simulink model "Heart_3D"  (R2024b)
settings: configuration reference "MasterConfig" (kept outside this file)
model workspace (MAT data in the model file):
  C_1 = 1
  C_10 = 23
  C_11 = 23
  C_12 = 23
  C_13 = 23
  C_14 = 23
  C_15 = 23
  C_16 = 23
  C_17 = 23
  C_18 = 23
  C_19 = 23
  C_2 = 1
  C_20 = 23
  C_21 = 23
  C_22 = 23
  C_23 = 2
  C_24 = 2
  C_25 = 2
  C_26 = 23
  C_27 = 23
  C_28 = 23
  C_29 = 23
  C_3 = 1
  C_30 = 50
  C_31 = 23
  C_32 = 23
  C_33 = 50
  C_34 = 23
  C_35 = 50
  C_36 = 23
  C_37 = 50
  C_38 = 50
  C_39 = 50
  C_4 = 1
  C_40 = 50
  C_41 = 50
  C_42 = 50
  C_43 = 50
  C_44 = 50
  C_45 = 23
  C_46 = 23
  C_47 = 23
  C_48 = 50
  C_49 = 50
  C_5 = 23
  C_50 = 23
  C_51 = 23
  C_52 = 23
  C_53 = 50
  C_54 = 50
  C_6 = 23
  C_7 = 23
  C_8 = 23
  C_9 = 23
  l_1 = 4.01400326634
  l_10 = 14.0362958077
  l_11 = 18.1950322891
  l_12 = 33.9599764429
  l_13 = 10
  l_14 = 8.0399004969
  l_15 = 12.0066648158
  l_16 = 7.69415362467
  l_17 = 5.21536192416
  l_18 = 5.65685424949
  l_19 = 13.8852439662
  l_2 = 3.2
  l_20 = 47.0387074652
  l_21 = 27.273430294
  l_22 = 13.8621787609
  l_23 = 18.6761880479
  l_24 = 12.8249756335
  l_25 = 15.879546593
  l_26 = 28.9689488936
  l_27 = 29.8073816361
  l_28 = 34.0352758179
  l_29 = 7.37563556583
  l_3 = 3.50907395191
  l_30 = 3.68781778292
  l_31 = 46.1042297409
  l_32 = 30.615028989
  l_33 = 7.51531769122
  l_34 = 7.47261667691
  l_35 = 3.73630833845
  l_36 = 36.7151195014
  l_37 = 16.1058995402
  l_38 = 48.7360236376
  l_39 = 48.8364617883
  l_4 = 4.54875807227
  l_40 = 41.4154560521
  l_41 = 37.7878287283
  l_42 = 44.689148571
  l_43 = 22.9120055866
  l_44 = 23.4401365184
  l_45 = 42.4264068712
  l_46 = 5
  l_47 = 8
  l_48 = 31.4273766007
  l_49 = 41.5788407727
  l_5 = 1.6986923075
  l_50 = 31.5569326773
  l_51 = 3
  l_52 = 3
  l_53 = 51.8478543433
  l_54 = 31.5569326773
  l_6 = 44.1540359298
  l_7 = 2.68208873828
  l_8 = 12.8
  l_9 = 4.53184289225
  xi_1 = 54.2
  xi_10 = 56.6
  xi_11 = 52.36
  xi_12 = 45
  xi_13 = 66.2
  xi_14 = 66.2
  xi_15 = 60.2
  xi_16 = 60.6
  xi_17 = 67
  xi_18 = 67.4
  xi_19 = 70.2
  xi_2 = 54.2
  xi_20 = 79.4
  xi_21 = 98.2
  xi_22 = 125.4
  xi_23 = 68.2
  xi_24 = 81.8
  xi_25 = 94.6
  xi_26 = 105
  xi_27 = 105
  xi_28 = 121.8
  xi_29 = 153
  xi_3 = 54.2
  xi_30 = 157.8
  xi_31 = 157.8
  xi_32 = 127.8
  xi_33 = 127.8
  xi_34 = 157
  xi_35 = 164.2
  xi_36 = 164.2
  xi_37 = 160.2
  xi_38 = 160.2
  xi_39 = 160.2
  xi_4 = 54.2
  xi_40 = 167.8
  xi_41 = 167.8
  xi_42 = 114.6
  xi_43 = 114.6
  xi_44 = 83
  xi_45 = 112.2
  xi_46 = 112.2
  xi_47 = 75
  xi_48 = 101.8
  xi_49 = 131
  xi_5 = 57.8666666667
  xi_50 = 159.4
  xi_51 = 159.4
  xi_52 = 143.4
  xi_53 = 112.2
  xi_54 = 162.4
  xi_6 = 57.8666666667
  xi_7 = 57.4
  xi_8 = 57.4
  xi_9 = 56.6
  xj_1 = 57.8666666667
  xj_10 = 66.2
  xj_11 = 45
  xj_12 = 53.8
  xj_13 = 60.2
  xj_14 = 67
  xj_15 = 60.6
  xj_16 = 68.2
  xj_17 = 67.4
  xj_18 = 68.2
  xj_19 = 79.4
  xj_2 = 57.4
  xj_20 = 118.6
  xj_21 = 125.4
  xj_22 = 135.4
  xj_23 = 81.8
  xj_24 = 94.6
  xj_25 = 105
  xj_26 = 121.8
  xj_27 = 127.8
  xj_28 = 153
  xj_29 = 157.8
  xj_3 = 56.6
  xj_30 = 160.2
  xj_31 = 112.2
  xj_32 = 157
  xj_33 = 131
  xj_34 = 164.2
  xj_35 = 167.8
  xj_36 = 159.4
  xj_37 = 167.8
  xj_38 = 114.6
  xj_39 = 112.2
  xj_4 = 52.36
  xj_40 = 131
  xj_41 = 162.4
  xj_42 = 83
  xj_43 = 131
  xj_44 = 101.8
  xj_45 = 75
  xj_46 = 112.2
  xj_47 = 67
  xj_48 = 125
  xj_49 = 101.8
  xj_5 = 57.4
  xj_50 = 143.4
  xj_51 = 162.4
  xj_52 = 146.4
  xj_53 = 67
  xj_54 = 146.4
  xj_6 = 98.2
  xj_7 = 56.6
  xj_8 = 70.2
  xj_9 = 52.36
  yi_1 = 118.2
  yi_10 = 115.64
  yi_11 = 114.04
  yi_12 = 97.4
  yi_13 = 105.4
  yi_14 = 105.4
  yi_15 = 97.4
  yi_16 = 85.4
  yi_17 = 97.4
  yi_18 = 92.2
  yi_19 = 118.2
  yi_2 = 118.2
  yi_20 = 107.8
  yi_21 = 137.8
  yi_22 = 139.8
  yi_23 = 86.6
  yi_24 = 99.4
  yi_25 = 100.2
  yi_26 = 88.2
  yi_27 = 88.2
  yi_28 = 64.6
  yi_29 = 51
  yi_3 = 118.2
  yi_30 = 45.4
  yi_31 = 45.4
  yi_32 = 69
  yi_33 = 69
  yi_34 = 59.8
  yi_35 = 57.8
  yi_36 = 57.8
  yi_37 = 42.6
  yi_38 = 42.6
  yi_39 = 42.6
  yi_4 = 118.2
  yi_40 = 56.8
  yi_41 = 56.8
  yi_42 = 59.8
  yi_43 = 59.8
  yi_44 = 91.4
  yi_45 = 38.6
  yi_46 = 38.6
  yi_47 = 59
  yi_48 = 105.4
  yi_49 = 75.8
  yi_5 = 119.833333333
  yi_50 = 94.2
  yi_51 = 94.2
  yi_52 = 121.4
  yi_53 = 33.6
  yi_54 = 94.2
  yi_6 = 119.833333333
  yi_7 = 118.2
  yi_8 = 118.2
  yi_9 = 115.64
  yj_1 = 119.833333333
  yj_10 = 105.4
  yj_11 = 97.4
  yj_12 = 64.6
  yj_13 = 97.4
  yj_14 = 97.4
  yj_15 = 85.4
  yj_16 = 86.6
  yj_17 = 92.2
  yj_18 = 86.6
  yj_19 = 107.8
  yj_2 = 118.2
  yj_20 = 133.8
  yj_21 = 139.8
  yj_22 = 130.2
  yj_23 = 99.4
  yj_24 = 100.2
  yj_25 = 88.2
  yj_26 = 64.6
  yj_27 = 69
  yj_28 = 51
  yj_29 = 45.4
  yj_3 = 115.64
  yj_30 = 42.6
  yj_31 = 38.6
  yj_32 = 59.8
  yj_33 = 75.8
  yj_34 = 57.8
  yj_35 = 56.8
  yj_36 = 94.2
  ... (+132 more variables)
undefined symbols (not defined in the file or in its folder): HeartCfg, Leads
(part 2 of 2)

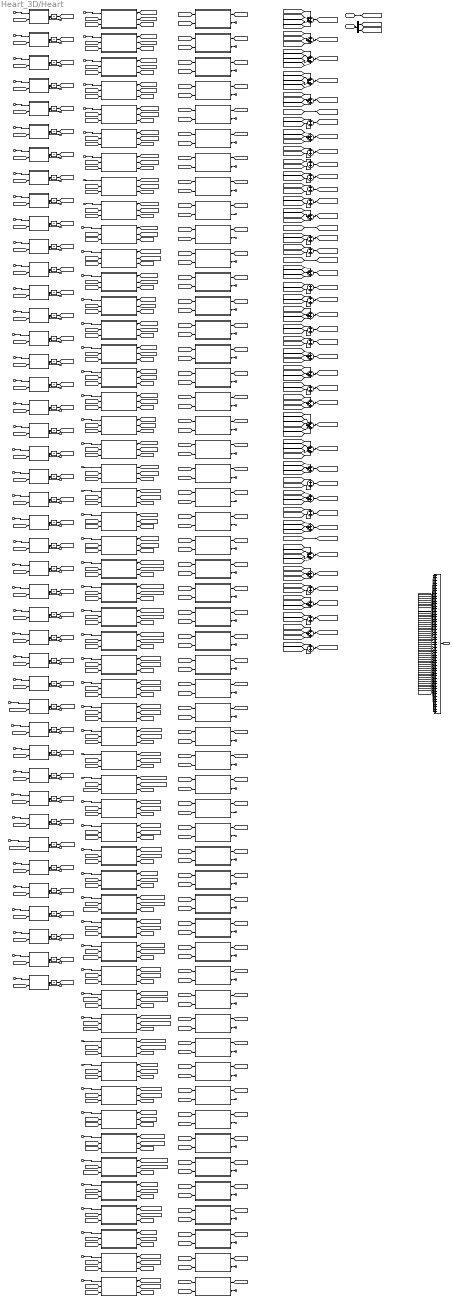
== system Heart_3D/Heart ==
  cfg_SA : Inport  PortName=cfg  Element=SA
  cfg_SA_a : Inport  PortName=cfg  Element=SA_a
  cfg_SA_b : Inport  PortName=cfg  Element=SA_b
  cfg_SA_c : Inport  PortName=cfg  Element=SA_c
  cfg_SA_d : Inport  PortName=cfg  Element=SA_d
  cfg_CT : Inport  PortName=cfg  Element=CT
  cfg_CT_a : Inport  PortName=cfg  Element=CT_a
  cfg_OS : Inport  PortName=cfg  Element=OS
  cfg_RE : Inport  PortName=cfg  Element=RE
  cfg_LNB : Inport  PortName=cfg  Element=LNB
  cfg_TC_f : Inport  PortName=cfg  Element=TC_f
  cfg_CN : Inport  PortName=cfg  Element=CN
  cfg_RA_a : Inport  PortName=cfg  Element=RA_a
  cfg_RA : Inport  PortName=cfg  Element=RA
  cfg_CS_LA : Inport  PortName=cfg  Element=CS_LA
  cfg_Bach : Inport  PortName=cfg  Element=Bach
  cfg_LA_a : Inport  PortName=cfg  Element=LA_a
  cfg_LA : Inport  PortName=cfg  Element=LA
  cfg_BH : Inport  PortName=cfg  Element=BH
  cfg_His_p : Inport  PortName=cfg  Element=His_p
  cfg_His_m : Inport  PortName=cfg  Element=His_m
  cfg_His_d : Inport  PortName=cfg  Element=His_d
  cfg_RBB_m : Inport  PortName=cfg  Element=RBB_m
  cfg_RBB : Inport  PortName=cfg  Element=RBB
  cfg_RBB_a : Inport  PortName=cfg  Element=RBB_a
  cfg_LBB_m : Inport  PortName=cfg  Element=LBB_m
  cfg_LBB : Inport  PortName=cfg  Element=LBB
  cfg_LBB_a : Inport  PortName=cfg  Element=LBB_a
  cfg_RVA : Inport  PortName=cfg  Element=RVA
  cfg_LVA : Inport  PortName=cfg  Element=LVA
  cfg_SEP_RV_m : Inport  PortName=cfg  Element=SEP_RV_m
  cfg_SEP_RV : Inport  PortName=cfg  Element=SEP_RV
  cfg_RV_m : Inport  PortName=cfg  Element=RV_m
  cfg_RV : Inport  PortName=cfg  Element=RV
  cfg_SEP_LV : Inport  PortName=cfg  Element=SEP_LV
  cfg_CS_LV : Inport  PortName=cfg  Element=CS_LV
  cfg_SEP_LV_m : Inport  PortName=cfg  Element=SEP_LV_m
  cfg_LV_m : Inport  PortName=cfg  Element=LV_m
  cfg_LV : Inport  PortName=cfg  Element=LV
  cfg_RV_mm : Inport  PortName=cfg  Element=RV_mm
  cfg_RVm : Inport  PortName=cfg  Element=RVm
  cfg_LV_mm : Inport  PortName=cfg  Element=LV_mm
  cfg_LVm : Inport  PortName=cfg  Element=LVm
  cfgPath_1_2 : Inport  PortName=cfg  Element=path_1
  cfgPath_1_3 : Inport  PortName=cfg  Element=path_2
  cfgPath_1_4 : Inport  PortName=cfg  Element=path_3
  cfgPath_1_5 : Inport  PortName=cfg  Element=path_4
  cfgPath_2_3 : Inport  PortName=cfg  Element=path_5
  cfgPath_2_16 : Inport  PortName=cfg  Element=path_6
  cfgPath_3_4 : Inport  PortName=cfg  Element=path_7
  cfgPath_3_13 : Inport  PortName=cfg  Element=path_8
  cfgPath_4_5 : Inport  PortName=cfg  Element=path_9
  cfgPath_4_8 : Inport  PortName=cfg  Element=path_10
  cfgPath_5_7 : Inport  PortName=cfg  Element=path_11
  cfgPath_6_7 : Inport  PortName=cfg  Element=path_12
  cfgPath_8_9 : Inport  PortName=cfg  Element=path_13
  cfgPath_8_11 : Inport  PortName=cfg  Element=path_14
  cfgPath_9_10 : Inport  PortName=cfg  Element=path_15
  cfgPath_10_19 : Inport  PortName=cfg  Element=path_16
  cfgPath_11_12 : Inport  PortName=cfg  Element=path_17
  cfgPath_12_19 : Inport  PortName=cfg  Element=path_18
  cfgPath_13_14 : Inport  PortName=cfg  Element=path_19
  cfgPath_14_15 : Inport  PortName=cfg  Element=path_20
  cfgPath_16_17 : Inport  PortName=cfg  Element=path_21
  cfgPath_17_18 : Inport  PortName=cfg  Element=path_22
  cfgPath_19_20 : Inport  PortName=cfg  Element=path_23
  cfgPath_20_21 : Inport  PortName=cfg  Element=path_24
  cfgPath_21_22 : Inport  PortName=cfg  Element=path_25
  cfgPath_22_23 : Inport  PortName=cfg  Element=path_26
  cfgPath_22_26 : Inport  PortName=cfg  Element=path_27
  cfgPath_23_24 : Inport  PortName=cfg  Element=path_28
  cfgPath_24_25 : Inport  PortName=cfg  Element=path_29
  cfgPath_25_29 : Inport  PortName=cfg  Element=path_30
  cfgPath_25_33 : Inport  PortName=cfg  Element=path_31
  cfgPath_26_27 : Inport  PortName=cfg  Element=path_32
  cfgPath_26_37 : Inport  PortName=cfg  Element=path_33
  cfgPath_27_28 : Inport  PortName=cfg  Element=path_34
  cfgPath_28_30 : Inport  PortName=cfg  Element=path_35
  cfgPath_28_38 : Inport  PortName=cfg  Element=path_36
  cfgPath_29_30 : Inport  PortName=cfg  Element=path_37
  cfgPath_29_31 : Inport  PortName=cfg  Element=path_38
  cfgPath_29_40 : Inport  PortName=cfg  Element=path_39
  cfgPath_30_37 : Inport  PortName=cfg  Element=path_40
  cfgPath_30_42 : Inport  PortName=cfg  Element=path_41
  cfgPath_31_32 : Inport  PortName=cfg  Element=path_42
  cfgPath_31_37 : Inport  PortName=cfg  Element=path_43
  cfgPath_32_35 : Inport  PortName=cfg  Element=path_44
  cfgPath_33_34 : Inport  PortName=cfg  Element=path_45
  cfgPath_33_40 : Inport  PortName=cfg  Element=path_46
  cfgPath_34_41 : Inport  PortName=cfg  Element=path_47
  cfgPath_35_36 : Inport  PortName=cfg  Element=path_48
  cfgPath_35_37 : Inport  PortName=cfg  Element=path_49
  cfgPath_38_39 : Inport  PortName=cfg  Element=path_50
  cfgPath_38_42 : Inport  PortName=cfg  Element=path_51
  cfgPath_39_43 : Inport  PortName=cfg  Element=path_52
  cfgPath_40_41 : Inport  PortName=cfg  Element=path_53
  cfgPath_42_43 : Inport  PortName=cfg  Element=path_54
  Leads : Inport  Port=2
  Pace : Inport  Port=3
  BH : ModelReference  ModelNameDialog=Node_NM  ModelReferenceVersion=1.97
  BH_His_p : ModelReference  ModelNameDialog=Path_model  ParameterArgumentNames=l  ParameterArgumentValues=l_23  UsingDefaultArgumentValue=0  ModelReferenceVersion=1.109
  BH_His_p_probe : ModelReference  ModelNameDialog=Electrode  UsingDefaultArgumentValue=0,0,0,0,0,0,0  ModelReferenceVersion=1.84
  Bach : ModelReference  ModelNameDialog=Node_M  ModelReferenceVersion=1.111
  Bach_LA_a : ModelReference  ModelNameDialog=Path_model  ParameterArgumentNames=l  ParameterArgumentValues=l_21  UsingDefaultArgumentValue=0  ModelReferenceVersion=1.109
  Bach_LA_a_probe : ModelReference  ModelNameDialog=Electrode  UsingDefaultArgumentValue=0,0,0,0,0,0,0  ModelReferenceVersion=1.84
  CN : ModelReference  ModelNameDialog=Node_N  ModelReferenceVersion=1.119
  CN_BH : ModelReference  ModelNameDialog=Path_model  ParameterArgumentNames=l  ParameterArgumentValues=l_18  UsingDefaultArgumentValue=0  ModelReferenceVersion=1.109
  CN_BH_probe : ModelReference  ModelNameDialog=Electrode  UsingDefaultArgumentValue=0,0,0,0,0,0,0  ModelReferenceVersion=1.84
  CS_LA : ModelReference  ModelNameDialog=Node_NM  ModelReferenceVersion=1.97
  CS_LV : ModelReference  ModelNameDialog=Node_M  ModelReferenceVersion=1.111
  CT : ModelReference  ModelNameDialog=Node_M  ModelReferenceVersion=1.111
  CT_CT_a : ModelReference  ModelNameDialog=Path_model  ParameterArgumentNames=l  ParameterArgumentValues=l_12  UsingDefaultArgumentValue=0  ModelReferenceVersion=1.109
  CT_CT_a_probe : ModelReference  ModelNameDialog=Electrode  UsingDefaultArgumentValue=0,0,0,0,0,0,0  ModelReferenceVersion=1.84
  CT_a : ModelReference  ModelNameDialog=Node_NM  ModelReferenceVersion=1.97
  CellDelay_BH : UnitDelay  SampleTime=-1  HasFrameUpgradeWarning=on
  CellDelay_Bach : UnitDelay  SampleTime=-1  HasFrameUpgradeWarning=on
  CellDelay_CN : UnitDelay  SampleTime=-1  HasFrameUpgradeWarning=on
  CellDelay_CS_LA : UnitDelay  SampleTime=-1  HasFrameUpgradeWarning=on
  CellDelay_CS_LV : UnitDelay  SampleTime=-1  HasFrameUpgradeWarning=on
  CellDelay_CT : UnitDelay  SampleTime=-1  HasFrameUpgradeWarning=on
  CellDelay_CT_a : UnitDelay  SampleTime=-1  HasFrameUpgradeWarning=on
  CellDelay_His_d : UnitDelay  SampleTime=-1  HasFrameUpgradeWarning=on
  CellDelay_His_m : UnitDelay  SampleTime=-1  HasFrameUpgradeWarning=on
  CellDelay_His_p : UnitDelay  SampleTime=-1  HasFrameUpgradeWarning=on
  CellDelay_LA : UnitDelay  SampleTime=-1  HasFrameUpgradeWarning=on
  CellDelay_LA_a : UnitDelay  SampleTime=-1  HasFrameUpgradeWarning=on
  CellDelay_LBB : UnitDelay  SampleTime=-1  HasFrameUpgradeWarning=on
  CellDelay_LBB_a : UnitDelay  SampleTime=-1  HasFrameUpgradeWarning=on
  CellDelay_LBB_m : UnitDelay  SampleTime=-1  HasFrameUpgradeWarning=on
  CellDelay_LNB : UnitDelay  SampleTime=-1  HasFrameUpgradeWarning=on
  CellDelay_LV : UnitDelay  SampleTime=-1  HasFrameUpgradeWarning=on
  CellDelay_LVA : UnitDelay  SampleTime=-1  HasFrameUpgradeWarning=on
  CellDelay_LV_m : UnitDelay  SampleTime=-1  HasFrameUpgradeWarning=on
  CellDelay_LV_mm : UnitDelay  SampleTime=-1  HasFrameUpgradeWarning=on
  CellDelay_LVm : UnitDelay  SampleTime=-1  HasFrameUpgradeWarning=on
  CellDelay_OS : UnitDelay  SampleTime=-1  HasFrameUpgradeWarning=on
  CellDelay_RA : UnitDelay  SampleTime=-1  HasFrameUpgradeWarning=on
  CellDelay_RA_a : UnitDelay  SampleTime=-1  HasFrameUpgradeWarning=on
  CellDelay_RBB : UnitDelay  SampleTime=-1  HasFrameUpgradeWarning=on
  CellDelay_RBB_a : UnitDelay  SampleTime=-1  HasFrameUpgradeWarning=on
  CellDelay_RBB_m : UnitDelay  SampleTime=-1  HasFrameUpgradeWarning=on
  CellDelay_RE : UnitDelay  SampleTime=-1  HasFrameUpgradeWarning=on
  CellDelay_RV : UnitDelay  SampleTime=-1  HasFrameUpgradeWarning=on
  CellDelay_RVA : UnitDelay  SampleTime=-1  HasFrameUpgradeWarning=on
  CellDelay_RV_m : UnitDelay  SampleTime=-1  HasFrameUpgradeWarning=on
  CellDelay_RV_mm : UnitDelay  SampleTime=-1  HasFrameUpgradeWarning=on
  CellDelay_RVm : UnitDelay  SampleTime=-1  HasFrameUpgradeWarning=on
  CellDelay_SA : UnitDelay  SampleTime=-1  HasFrameUpgradeWarning=on
  CellDelay_SA_a : UnitDelay  SampleTime=-1  HasFrameUpgradeWarning=on
  CellDelay_SA_b : UnitDelay  SampleTime=-1  HasFrameUpgradeWarning=on
  CellDelay_SA_c : UnitDelay  SampleTime=-1  HasFrameUpgradeWarning=on
  CellDelay_SA_d : UnitDelay  SampleTime=-1  HasFrameUpgradeWarning=on
  CellDelay_SEP_LV : UnitDelay  SampleTime=-1  HasFrameUpgradeWarning=on
  CellDelay_SEP_LV_m : UnitDelay  SampleTime=-1  HasFrameUpgradeWarning=on
  CellDelay_SEP_RV : UnitDelay  SampleTime=-1  HasFrameUpgradeWarning=on
  CellDelay_SEP_RV_m : UnitDelay  SampleTime=-1  HasFrameUpgradeWarning=on
  CellDelay_TC_f : UnitDelay  SampleTime=-1  HasFrameUpgradeWarning=on
  EGMs_Sum : Sum  Inputs=++++++++++++++++++++++++++++++++++++++++++++++++++++++
  His_d : ModelReference  ModelNameDialog=Node_NM  ModelReferenceVersion=1.97
  His_d_LBB_m : ModelReference  ModelNameDialog=Path_model  ParameterArgumentNames=l  ParameterArgumentValues=l_27  UsingDefaultArgumentValue=0  ModelReferenceVersion=1.109
  His_d_LBB_m_probe : ModelReference  ModelNameDialog=Electrode  UsingDefaultArgumentValue=0,0,0,0,0,0,0  ModelReferenceVersion=1.84
  His_d_RBB_m : ModelReference  ModelNameDialog=Path_model  ParameterArgumentNames=l  ParameterArgumentValues=l_26  UsingDefaultArgumentValue=0  ModelReferenceVersion=1.109
  His_d_RBB_m_probe : ModelReference  ModelNameDialog=Electrode  UsingDefaultArgumentValue=0,0,0,0,0,0,0  ModelReferenceVersion=1.84
  His_m : ModelReference  ModelNameDialog=Node_NM  ModelReferenceVersion=1.97
  His_m_His_d : ModelReference  ModelNameDialog=Path_model  ParameterArgumentNames=l  ParameterArgumentValues=l_25  UsingDefaultArgumentValue=0  ModelReferenceVersion=1.109
  His_m_His_d_probe : ModelReference  ModelNameDialog=Electrode  UsingDefaultArgumentValue=0,0,0,0,0,0,0  ModelReferenceVersion=1.84
  His_p : ModelReference  ModelNameDialog=Node_NM  ModelReferenceVersion=1.97
  His_p_His_m : ModelReference  ModelNameDialog=Path_model  ParameterArgumentNames=l  ParameterArgumentValues=l_24  UsingDefaultArgumentValue=0  ModelReferenceVersion=1.109
  His_p_His_m_probe : ModelReference  ModelNameDialog=Electrode  UsingDefaultArgumentValue=0,0,0,0,0,0,0  ModelReferenceVersion=1.84
  LA : ModelReference  ModelNameDialog=Node_M  ModelReferenceVersion=1.111
  LA_a : ModelReference  ModelNameDialog=Node_M  ModelReferenceVersion=1.111
  LA_a_LA : ModelReference  ModelNameDialog=Path_model  ParameterArgumentNames=l  ParameterArgumentValues=l_22  UsingDefaultArgumentValue=0  ModelReferenceVersion=1.109
  LA_a_LA_probe : ModelReference  ModelNameDialog=Electrode  UsingDefaultArgumentValue=0,0,0,0,0,0,0  ModelReferenceVersion=1.84
  LBB : ModelReference  ModelNameDialog=Node_NM  ModelReferenceVersion=1.97
  LBB_LBB_a : ModelReference  ModelNameDialog=Path_model  ParameterArgumentNames=l  ParameterArgumentValues=l_34  UsingDefaultArgumentValue=0  ModelReferenceVersion=1.109
  LBB_LBB_a_probe : ModelReference  ModelNameDialog=Electrode  UsingDefaultArgumentValue=0,0,0,0,0,0,0  ModelReferenceVersion=1.84
  LBB_a : ModelReference  ModelNameDialog=Node_NM  ModelReferenceVersion=1.97
  LBB_a_LVA : ModelReference  ModelNameDialog=Path_model  ParameterArgumentNames=l  ParameterArgumentValues=l_35  UsingDefaultArgumentValue=0  ModelReferenceVersion=1.109
  LBB_a_LVA_probe : ModelReference  ModelNameDialog=Electrode  UsingDefaultArgumentValue=0,0,0,0,0,0,0  ModelReferenceVersion=1.84
  LBB_a_LV_m : ModelReference  ModelNameDialog=Path_model  ParameterArgumentNames=l  ParameterArgumentValues=l_36  UsingDefaultArgumentValue=0  ModelReferenceVersion=1.109
  LBB_a_LV_m_probe : ModelReference  ModelNameDialog=Electrode  UsingDefaultArgumentValue=0,0,0,0,0,0,0  ModelReferenceVersion=1.84
  LBB_m : ModelReference  ModelNameDialog=Node_NM  ModelReferenceVersion=1.97
  LBB_m_LBB : ModelReference  ModelNameDialog=Path_model  ParameterArgumentNames=l  ParameterArgumentValues=l_32  UsingDefaultArgumentValue=0  ModelReferenceVersion=1.109
  LBB_m_LBB_probe : ModelReference  ModelNameDialog=Electrode  UsingDefaultArgumentValue=0,0,0,0,0,0,0  ModelReferenceVersion=1.84
  LBB_m_SEP_LV_m : ModelReference  ModelNameDialog=Path_model  ParameterArgumentNames=l  ParameterArgumentValues=l_33  UsingDefaultArgumentValue=0  ModelReferenceVersion=1.109
  LBB_m_SEP_LV_m_probe : ModelReference  ModelNameDialog=Electrode  UsingDefaultArgumentValue=0,0,0,0,0,0,0  ModelReferenceVersion=1.84
  LNB : ModelReference  ModelNameDialog=Node_NM  ModelReferenceVersion=1.97
  LNB_BH : ModelReference  ModelNameDialog=Path_model  ParameterArgumentNames=l  ParameterArgumentValues=l_16  UsingDefaultArgumentValue=0  ModelReferenceVersion=1.109
  LNB_BH_probe : ModelReference  ModelNameDialog=Electrode  UsingDefaultArgumentValue=0,0,0,0,0,0,0  ModelReferenceVersion=1.84
  LV : ModelReference  ModelNameDialog=Node_NM  ModelReferenceVersion=1.97
  LVA : ModelReference  ModelNameDialog=Node_M  ModelReferenceVersion=1.111
  LVA_LV_mm : ModelReference  ModelNameDialog=Path_model  ParameterArgumentNames=l  ParameterArgumentValues=l_41  UsingDefaultArgumentValue=0  ModelReferenceVersion=1.109
  LVA_LV_mm_probe : ModelReference  ModelNameDialog=Electrode  UsingDefaultArgumentValue=0,0,0,0,0,0,0  ModelReferenceVersion=1.84
  LVA_SEP_LV_m : ModelReference  ModelNameDialog=Path_model  ParameterArgumentNames=l  ParameterArgumentValues=l_40  UsingDefaultArgumentValue=0  ModelReferenceVersion=1.109
  LVA_SEP_LV_m_probe : ModelReference  ModelNameDialog=Electrode  UsingDefaultArgumentValue=0,0,0,0,0,0,0  ModelReferenceVersion=1.84
  LV_LVm : ModelReference  ModelNameDialog=Path_model  ParameterArgumentNames=l  ParameterArgumentValues=l_52  UsingDefaultArgumentValue=0  ModelReferenceVersion=1.109
  LV_LVm_probe : ModelReference  ModelNameDialog=Electrode  UsingDefaultArgumentValue=0,0,0,0,0,0,0  ModelReferenceVersion=1.84
  LV_m : ModelReference  ModelNameDialog=Node_NM  ModelReferenceVersion=1.97
  LV_m_LV : ModelReference  ModelNameDialog=Path_model  ParameterArgumentNames=l  ParameterArgumentValues=l_50  UsingDefaultArgumentValue=0  ModelReferenceVersion=1.109
  LV_m_LV_mm : ModelReference  ModelNameDialog=Path_model  ParameterArgumentNames=l  ParameterArgumentValues=l_51  UsingDefaultArgumentValue=0  ModelReferenceVersion=1.109
  LV_m_LV_mm_probe : ModelReference  ModelNameDialog=Electrode  UsingDefaultArgumentValue=0,0,0,0,0,0,0  ModelReferenceVersion=1.84
  LV_m_LV_probe : ModelReference  ModelNameDialog=Electrode  UsingDefaultArgumentValue=0,0,0,0,0,0,0  ModelReferenceVersion=1.84
  LV_mm : ModelReference  ModelNameDialog=Node_M  ModelReferenceVersion=1.111
  LV_mm_LVm : ModelReference  ModelNameDialog=Path_model  ParameterArgumentNames=l  ParameterArgumentValues=l_54  UsingDefaultArgumentValue=0  ModelReferenceVersion=1.109
  LV_mm_LVm_probe : ModelReference  ModelNameDialog=Electrode  UsingDefaultArgumentValue=0,0,0,0,0,0,0  ModelReferenceVersion=1.84
  LVm : ModelReference  ModelNameDialog=Node_M  ModelReferenceVersion=1.111
  Node10_OR : Sum  Inputs=2
  Node11_OR : Sum  Inputs=2
  Node12_OR : Sum  Inputs=2
  Node13_OR : Sum  Inputs=2
  Node14_OR : Sum  Inputs=3
  Node16_OR : Sum  Inputs=2
  Node17_OR : Sum  Inputs=2
  Node19_OR : Sum  Inputs=3
  Node1_OR : Sum  Inputs=4
  Node20_OR : Sum  Inputs=2
  Node21_OR : Sum  Inputs=2
  Node22_OR : Sum  Inputs=3
  Node23_OR : Sum  Inputs=2
  Node24_OR : Sum  Inputs=2
  Node25_OR : Sum  Inputs=3
  Node26_OR : Sum  Inputs=3
  Node27_OR : Sum  Inputs=2
  Node28_OR : Sum  Inputs=3
  Node29_OR : Sum  Inputs=5
  Node2_OR : Sum  Inputs=3
  Node30_OR : Sum  Inputs=4
  Node31_OR : Sum  Inputs=3
  Node32_OR : Sum  Inputs=2
  Node33_OR : Sum  Inputs=3
  Node34_OR : Sum  Inputs=2
  Node35_OR : Sum  Inputs=3
  Node37_OR : Sum  Inputs=4
  Node38_OR : Sum  Inputs=3
  Node39_OR : Sum  Inputs=2
  Node3_OR : Sum  Inputs=4
  Node40_OR : Sum  Inputs=3
  Node41_OR : Sum  Inputs=2
  Node42_OR : Sum  Inputs=3
  Node43_OR : Sum  Inputs=2
  Node4_OR : Sum  Inputs=4
  Node5_OR : Sum  Inputs=3
  Node7_OR : Sum  Inputs=2
  Node8_OR : Sum  Inputs=3
  Node9_OR : Sum  Inputs=2
  OS : ModelReference  ModelNameDialog=Node_NM  ModelReferenceVersion=1.97
  OS_RE : ModelReference  ModelNameDialog=Path_model  ParameterArgumentNames=l  ParameterArgumentValues=l_13  UsingDefaultArgumentValue=0  ModelReferenceVersion=1.109
  OS_RE_probe : ModelReference  ModelNameDialog=Electrode  UsingDefaultArgumentValue=0,0,0,0,0,0,0  ModelReferenceVersion=1.84
  OS_TC_f : ModelReference  ModelNameDialog=Path_model  ParameterArgumentNames=l  ParameterArgumentValues=l_14  UsingDefaultArgumentValue=0  ModelReferenceVersion=1.109
  OS_TC_f_probe : ModelReference  ModelNameDialog=Electrode  UsingDefaultArgumentValue=0,0,0,0,0,0,0  ModelReferenceVersion=1.84
  Pacing : Demux  Outputs=2
  RA : ModelReference  ModelNameDialog=Node_M  ModelReferenceVersion=1.111
  RA_CS_LA : ModelReference  ModelNameDialog=Path_model  ParameterArgumentNames=l  ParameterArgumentValues=l_20  UsingDefaultArgumentValue=0  ModelReferenceVersion=1.109
  RA_CS_LA_probe : ModelReference  ModelNameDialog=Electrode  UsingDefaultArgumentValue=0,0,0,0,0,0,0  ModelReferenceVersion=1.84
  RA_a : ModelReference  ModelNameDialog=Node_M  ModelReferenceVersion=1.111
  RA_a_RA : ModelReference  ModelNameDialog=Path_model  ParameterArgumentNames=l  ParameterArgumentValues=l_19  UsingDefaultArgumentValue=0  ModelReferenceVersion=1.109
  RA_a_RA_probe : ModelReference  ModelNameDialog=Electrode  UsingDefaultArgumentValue=0,0,0,0,0,0,0  ModelReferenceVersion=1.84
  RBB : ModelReference  ModelNameDialog=Node_NM  ModelReferenceVersion=1.97
  RBB_RBB_a : ModelReference  ModelNameDialog=Path_model  ParameterArgumentNames=l  ParameterArgumentValues=l_29  UsingDefaultArgumentValue=0  ModelReferenceVersion=1.109
  RBB_RBB_a_probe : ModelReference  ModelNameDialog=Electrode  UsingDefaultArgumentValue=0,0,0,0,0,0,0  ModelReferenceVersion=1.84
  RBB_a : ModelReference  ModelNameDialog=Node_NM  ModelReferenceVersion=1.97
  RBB_a_RVA : ModelReference  ModelNameDialog=Path_model  ParameterArgumentNames=l  ParameterArgumentValues=l_30  UsingDefaultArgumentValue=0  ModelReferenceVersion=1.109
  RBB_a_RVA_probe : ModelReference  ModelNameDialog=Electrode  UsingDefaultArgumentValue=0,0,0,0,0,0,0  ModelReferenceVersion=1.84
  RBB_a_RV_m : ModelReference  ModelNameDialog=Path_model  ParameterArgumentNames=l  ParameterArgumentValues=l_31  UsingDefaultArgumentValue=0  ModelReferenceVersion=1.109
  RBB_a_RV_m_probe : ModelReference  ModelNameDialog=Electrode  UsingDefaultArgumentValue=0,0,0,0,0,0,0  ModelReferenceVersion=1.84
  RBB_m : ModelReference  ModelNameDialog=Node_NM  ModelReferenceVersion=1.97
  RBB_m_RBB : ModelReference  ModelNameDialog=Path_model  ParameterArgumentNames=l  ParameterArgumentValues=l_28  UsingDefaultArgumentValue=0  ModelReferenceVersion=1.109
  RBB_m_RBB_probe : ModelReference  ModelNameDialog=Electrode  UsingDefaultArgumentValue=0,0,0,0,0,0,0  ModelReferenceVersion=1.84
  RE : ModelReference  ModelNameDialog=Node_N  ModelReferenceVersion=1.119
  RE_LNB : ModelReference  ModelNameDialog=Path_model  ParameterArgumentNames=l  ParameterArgumentValues=l_15  UsingDefaultArgumentValue=0  ModelReferenceVersion=1.109
  RE_LNB_probe : ModelReference  ModelNameDialog=Electrode  UsingDefaultArgumentValue=0,0,0,0,0,0,0  ModelReferenceVersion=1.84
  RV : ModelReference  ModelNameDialog=Node_NM  ModelReferenceVersion=1.97
  RVA : ModelReference  ModelNameDialog=Node_M  ModelReferenceVersion=1.111
  RVA_LVA : ModelReference  ModelNameDialog=Path_model  ParameterArgumentNames=l  ParameterArgumentValues=l_37  UsingDefaultArgumentValue=0  ModelReferenceVersion=1.109
  RVA_LVA_probe : ModelReference  ModelNameDialog=Electrode  UsingDefaultArgumentValue=0,0,0,0,0,0,0  ModelReferenceVersion=1.84
  RVA_RV_mm : ModelReference  ModelNameDialog=Path_model  ParameterArgumentNames=l  ParameterArgumentValues=l_39  UsingDefaultArgumentValue=0  ModelReferenceVersion=1.109
  RVA_RV_mm_probe : ModelReference  ModelNameDialog=Electrode  UsingDefaultArgumentValue=0,0,0,0,0,0,0  ModelReferenceVersion=1.84
  RVA_SEP_RV_m : ModelReference  ModelNameDialog=Path_model  ParameterArgumentNames=l  ParameterArgumentValues=l_38  UsingDefaultArgumentValue=0  ModelReferenceVersion=1.109
  RVA_SEP_RV_m_probe : ModelReference  ModelNameDialog=Electrode  UsingDefaultArgumentValue=0,0,0,0,0,0,0  ModelReferenceVersion=1.84
  RV_RVm : ModelReference  ModelNameDialog=Path_model  ParameterArgumentNames=l  ParameterArgumentValues=l_47  UsingDefaultArgumentValue=0  ModelReferenceVersion=1.109
  RV_RVm_probe : ModelReference  ModelNameDialog=Electrode  UsingDefaultArgumentValue=0,0,0,0,0,0,0  ModelReferenceVersion=1.84
  RV_m : ModelReference  ModelNameDialog=Node_NM  ModelReferenceVersion=1.97
  RV_m_RV : ModelReference  ModelNameDialog=Path_model  ParameterArgumentNames=l  ParameterArgumentValues=l_45  UsingDefaultArgumentValue=0  ModelReferenceVersion=1.109
  RV_m_RV_mm : ModelReference  ModelNameDialog=Path_model  ParameterArgumentNames=l  ParameterArgumentValues=l_46  UsingDefaultArgumentValue=0  ModelReferenceVersion=1.109
  RV_m_RV_mm_probe : ModelReference  ModelNameDialog=Electrode  UsingDefaultArgumentValue=0,0,0,0,0,0,0  ModelReferenceVersion=1.84
  RV_m_RV_probe : ModelReference  ModelNameDialog=Electrode  UsingDefaultArgumentValue=0,0,0,0,0,0,0  ModelReferenceVersion=1.84
  RV_mm : ModelReference  ModelNameDialog=Node_M  ModelReferenceVersion=1.111
  RV_mm_RVm : ModelReference  ModelNameDialog=Path_model  ParameterArgumentNames=l  ParameterArgumentValues=l_53  UsingDefaultArgumentValue=0  ModelReferenceVersion=1.109
  RV_mm_RVm_probe : ModelReference  ModelNameDialog=Electrode  UsingDefaultArgumentValue=0,0,0,0,0,0,0  ModelReferenceVersion=1.84
  RVm : ModelReference  ModelNameDialog=Node_M  ModelReferenceVersion=1.111
  SA : ModelReference  ModelNameDialog=Node_N  ModelReferenceVersion=1.119
  SA_SA_a : ModelReference  ModelNameDialog=Path_model  ParameterArgumentNames=l  ParameterArgumentValues=l_1  UsingDefaultArgumentValue=0  ModelReferenceVersion=1.109
  SA_SA_a_probe : ModelReference  ModelNameDialog=Electrode  UsingDefaultArgumentValue=0,0,0,0,0,0,0  ModelReferenceVersion=1.84
  SA_SA_b : ModelReference  ModelNameDialog=Path_model  ParameterArgumentNames=l  ParameterArgumentValues=l_2  UsingDefaultArgumentValue=0  ModelReferenceVersion=1.109
  SA_SA_b_probe : ModelReference  ModelNameDialog=Electrode  UsingDefaultArgumentValue=0,0,0,0,0,0,0  ModelReferenceVersion=1.84
  SA_SA_c : ModelReference  ModelNameDialog=Path_model  ParameterArgumentNames=l  ParameterArgumentValues=l_3  UsingDefaultArgumentValue=0  ModelReferenceVersion=1.109
  SA_SA_c_probe : ModelReference  ModelNameDialog=Electrode  UsingDefaultArgumentValue=0,0,0,0,0,0,0  ModelReferenceVersion=1.84
  SA_SA_d : ModelReference  ModelNameDialog=Path_model  ParameterArgumentNames=l  ParameterArgumentValues=l_4  UsingDefaultArgumentValue=0  ModelReferenceVersion=1.109
  SA_SA_d_probe : ModelReference  ModelNameDialog=Electrode  UsingDefaultArgumentValue=0,0,0,0,0,0,0  ModelReferenceVersion=1.84
  SA_a : ModelReference  ModelNameDialog=Node_M  ModelReferenceVersion=1.111
  SA_a_Bach : ModelReference  ModelNameDialog=Path_model  ParameterArgumentNames=l  ParameterArgumentValues=l_6  UsingDefaultArgumentValue=0  ModelReferenceVersion=1.109
  SA_a_Bach_probe : ModelReference  ModelNameDialog=Electrode  UsingDefaultArgumentValue=0,0,0,0,0,0,0  ModelReferenceVersion=1.84
  SA_a_SA_b : ModelReference  ModelNameDialog=Path_model  ParameterArgumentNames=l  ParameterArgumentValues=l_5  UsingDefaultArgumentValue=0  ModelReferenceVersion=1.109
  SA_a_SA_b_probe : ModelReference  ModelNameDialog=Electrode  UsingDefaultArgumentValue=0,0,0,0,0,0,0  ModelReferenceVersion=1.84
  SA_b : ModelReference  ModelNameDialog=Node_M  ModelReferenceVersion=1.111
  SA_b_RA_a : ModelReference  ModelNameDialog=Path_model  ParameterArgumentNames=l  ParameterArgumentValues=l_8  UsingDefaultArgumentValue=0  ModelReferenceVersion=1.109
  SA_b_RA_a_probe : ModelReference  ModelNameDialog=Electrode  UsingDefaultArgumentValue=0,0,0,0,0,0,0  ModelReferenceVersion=1.84
  SA_b_SA_c : ModelReference  ModelNameDialog=Path_model  ParameterArgumentNames=l  ParameterArgumentValues=l_7  UsingDefaultArgumentValue=0  ModelReferenceVersion=1.109
  SA_b_SA_c_probe : ModelReference  ModelNameDialog=Electrode  UsingDefaultArgumentValue=0,0,0,0,0,0,0  ModelReferenceVersion=1.84
  SA_c : ModelReference  ModelNameDialog=Node_M  ModelReferenceVersion=1.111
  SA_c_OS : ModelReference  ModelNameDialog=Path_model  ParameterArgumentNames=l  ParameterArgumentValues=l_10  UsingDefaultArgumentValue=0  ModelReferenceVersion=1.109
  SA_c_OS_probe : ModelReference  ModelNameDialog=Electrode  UsingDefaultArgumentValue=0,0,0,0,0,0,0  ModelReferenceVersion=1.84
  SA_c_SA_d : ModelReference  ModelNameDialog=Path_model  ParameterArgumentNames=l  ParameterArgumentValues=l_9  UsingDefaultArgumentValue=0  ModelReferenceVersion=1.109
  SA_c_SA_d_probe : ModelReference  ModelNameDialog=Electrode  UsingDefaultArgumentValue=0,0,0,0,0,0,0  ModelReferenceVersion=1.84
  SA_d : ModelReference  ModelNameDialog=Node_NM  ModelReferenceVersion=1.97
  SA_d_CT_a : ModelReference  ModelNameDialog=Path_model  ParameterArgumentNames=l  ParameterArgumentValues=l_11  UsingDefaultArgumentValue=0  ModelReferenceVersion=1.109
  SA_d_CT_a_probe : ModelReference  ModelNameDialog=Electrode  UsingDefaultArgumentValue=0,0,0,0,0,0,0  ModelReferenceVersion=1.84
  SEP_LV : ModelReference  ModelNameDialog=Node_M  ModelReferenceVersion=1.111
  SEP_LV_CS_LV : ModelReference  ModelNameDialog=Path_model  ParameterArgumentNames=l  ParameterArgumentValues=l_48  UsingDefaultArgumentValue=0  ModelReferenceVersion=1.109
  SEP_LV_CS_LV_probe : ModelReference  ModelNameDialog=Electrode  UsingDefaultArgumentValue=0,0,0,0,0,0,0  ModelReferenceVersion=1.84
  SEP_LV_SEP_LV_m : ModelReference  ModelNameDialog=Path_model  ParameterArgumentNames=l  ParameterArgumentValues=l_49  UsingDefaultArgumentValue=0  ModelReferenceVersion=1.109
  SEP_LV_SEP_LV_m_probe : ModelReference  ModelNameDialog=Electrode  UsingDefaultArgumentValue=0,0,0,0,0,0,0  ModelReferenceVersion=1.84
  SEP_LV_m : ModelReference  ModelNameDialog=Node_M  ModelReferenceVersion=1.111
  SEP_RV : ModelReference  ModelNameDialog=Node_M  ModelReferenceVersion=1.111
  SEP_RV_SEP_LV : ModelReference  ModelNameDialog=Path_model  ParameterArgumentNames=l  ParameterArgumentValues=l_44  UsingDefaultArgumentValue=0  ModelReferenceVersion=1.109
  SEP_RV_SEP_LV_probe : ModelReference  ModelNameDialog=Electrode  UsingDefaultArgumentValue=0,0,0,0,0,0,0  ModelReferenceVersion=1.84
  SEP_RV_m : ModelReference  ModelNameDialog=Node_M  ModelReferenceVersion=1.111
  SEP_RV_m_SEP_LV_m : ModelReference  ModelNameDialog=Path_model  ParameterArgumentNames=l  ParameterArgumentValues=l_43  UsingDefaultArgumentValue=0  ModelReferenceVersion=1.109
  SEP_RV_m_SEP_LV_m_probe : ModelReference  ModelNameDialog=Electrode  UsingDefaultArgumentValue=0,0,0,0,0,0,0  ModelReferenceVersion=1.84
  SEP_RV_m_SEP_RV : ModelReference  ModelNameDialog=Path_model  ParameterArgumentNames=l  ParameterArgumentValues=l_42  UsingDefaultArgumentValue=0  ModelReferenceVersion=1.109
  SEP_RV_m_SEP_RV_probe : ModelReference  ModelNameDialog=Electrode  UsingDefaultArgumentValue=0,0,0,0,0,0,0  ModelReferenceVersion=1.84
  TC_f : ModelReference  ModelNameDialog=Node_NM  ModelReferenceVersion=1.97
  TC_f_CN : ModelReference  ModelNameDialog=Path_model  ParameterArgumentNames=l  ParameterArgumentValues=l_17  UsingDefaultArgumentValue=0  ModelReferenceVersion=1.109
  TC_f_CN_probe : ModelReference  ModelNameDialog=Electrode  UsingDefaultArgumentValue=0,0,0,0,0,0,0  ModelReferenceVersion=1.84
  Cells_c_SA : Outport  PortName=Cells  Element=c_SA
  Cells_c_SA_a : Outport  PortName=Cells  Element=c_SA_a
  Cells_c_SA_b : Outport  PortName=Cells  Element=c_SA_b
  Cells_c_SA_c : Outport  PortName=Cells  Element=c_SA_c
  Cells_c_SA_d : Outport  PortName=Cells  Element=c_SA_d
  Cells_c_CT : Outport  PortName=Cells  Element=c_CT
  Cells_c_CT_a : Outport  PortName=Cells  Element=c_CT_a
  Cells_c_OS : Outport  PortName=Cells  Element=c_OS
  Cells_c_RE : Outport  PortName=Cells  Element=c_RE
  Cells_c_LNB : Outport  PortName=Cells  Element=c_LNB
  Cells_c_TC_f : Outport  PortName=Cells  Element=c_TC_f
  Cells_c_CN : Outport  PortName=Cells  Element=c_CN
  Cells_c_RA_a : Outport  PortName=Cells  Element=c_RA_a
  Cells_c_RA : Outport  PortName=Cells  Element=c_RA
  Cells_c_CS_LA : Outport  PortName=Cells  Element=c_CS_LA
  Cells_c_Bach : Outport  PortName=Cells  Element=c_Bach
  Cells_c_LA_a : Outport  PortName=Cells  Element=c_LA_a
  Cells_c_LA : Outport  PortName=Cells  Element=c_LA
  Cells_c_BH : Outport  PortName=Cells  Element=c_BH
  Cells_c_His_p : Outport  PortName=Cells  Element=c_His_p
  Cells_c_His_m : Outport  PortName=Cells  Element=c_His_m
  Cells_c_His_d : Outport  PortName=Cells  Element=c_His_d
  Cells_c_RBB_m : Outport  PortName=Cells  Element=c_RBB_m
  Cells_c_RBB : Outport  PortName=Cells  Element=c_RBB
  Cells_c_RBB_a : Outport  PortName=Cells  Element=c_RBB_a
  Cells_c_LBB_m : Outport  PortName=Cells  Element=c_LBB_m
  Cells_c_LBB : Outport  PortName=Cells  Element=c_LBB
  Cells_c_LBB_a : Outport  PortName=Cells  Element=c_LBB_a
  Cells_c_RVA : Outport  PortName=Cells  Element=c_RVA
  Cells_c_LVA : Outport  PortName=Cells  Element=c_LVA
  Cells_c_SEP_RV_m : Outport  PortName=Cells  Element=c_SEP_RV_m
  Cells_c_SEP_RV : Outport  PortName=Cells  Element=c_SEP_RV
  Cells_c_RV_m : Outport  PortName=Cells  Element=c_RV_m
  Cells_c_RV : Outport  PortName=Cells  Element=c_RV
  Cells_c_SEP_LV : Outport  PortName=Cells  Element=c_SEP_LV
  Cells_c_CS_LV : Outport  PortName=Cells  Element=c_CS_LV
  Cells_c_SEP_LV_m : Outport  PortName=Cells  Element=c_SEP_LV_m
  Cells_c_LV_m : Outport  PortName=Cells  Element=c_LV_m
  Cells_c_LV : Outport  PortName=Cells  Element=c_LV
  Cells_c_RV_mm : Outport  PortName=Cells  Element=c_RV_mm
  Cells_c_RVm : Outport  PortName=Cells  Element=c_RVm
  Cells_c_LV_mm : Outport  PortName=Cells  Element=c_LV_mm
  Cells_c_LVm : Outport  PortName=Cells  Element=c_LVm
  EGMs : Outport  Port=2
  waves_w_1 : Outport  Port=3  PortName=waves  Element=w_1
  waves_w_2 : Outport  Port=3  PortName=waves  Element=w_2
  waves_w_3 : Outport  Port=3  PortName=waves  Element=w_3
  waves_w_4 : Outport  Port=3  PortName=waves  Element=w_4
  waves_w_5 : Outport  Port=3  PortName=waves  Element=w_5
  waves_w_6 : Outport  Port=3  PortName=waves  Element=w_6
  waves_w_7 : Outport  Port=3  PortName=waves  Element=w_7
  waves_w_8 : Outport  Port=3  PortName=waves  Element=w_8
  waves_w_9 : Outport  Port=3  PortName=waves  Element=w_9
  waves_w_10 : Outport  Port=3  PortName=waves  Element=w_10
  waves_w_11 : Outport  Port=3  PortName=waves  Element=w_11
  waves_w_12 : Outport  Port=3  PortName=waves  Element=w_12
  waves_w_13 : Outport  Port=3  PortName=waves  Element=w_13
  waves_w_14 : Outport  Port=3  PortName=waves  Element=w_14
  waves_w_15 : Outport  Port=3  PortName=waves  Element=w_15
  waves_w_16 : Outport  Port=3  PortName=waves  Element=w_16
  waves_w_17 : Outport  Port=3  PortName=waves  Element=w_17
  waves_w_18 : Outport  Port=3  PortName=waves  Element=w_18
  waves_w_19 : Outport  Port=3  PortName=waves  Element=w_19
  waves_w_20 : Outport  Port=3  PortName=waves  Element=w_20
  waves_w_21 : Outport  Port=3  PortName=waves  Element=w_21
  waves_w_22 : Outport  Port=3  PortName=waves  Element=w_22
  waves_w_23 : Outport  Port=3  PortName=waves  Element=w_23
  waves_w_24 : Outport  Port=3  PortName=waves  Element=w_24
  waves_w_25 : Outport  Port=3  PortName=waves  Element=w_25
  waves_w_26 : Outport  Port=3  PortName=waves  Element=w_26
  waves_w_27 : Outport  Port=3  PortName=waves  Element=w_27
  waves_w_28 : Outport  Port=3  PortName=waves  Element=w_28
  waves_w_29 : Outport  Port=3  PortName=waves  Element=w_29
  waves_w_30 : Outport  Port=3  PortName=waves  Element=w_30
  waves_w_31 : Outport  Port=3  PortName=waves  Element=w_31
  waves_w_32 : Outport  Port=3  PortName=waves  Element=w_32
  waves_w_33 : Outport  Port=3  PortName=waves  Element=w_33
  waves_w_34 : Outport  Port=3  PortName=waves  Element=w_34
  waves_w_35 : Outport  Port=3  PortName=waves  Element=w_35
  waves_w_36 : Outport  Port=3  PortName=waves  Element=w_36
  waves_w_37 : Outport  Port=3  PortName=waves  Element=w_37
  waves_w_38 : Outport  Port=3  PortName=waves  Element=w_38
  waves_w_39 : Outport  Port=3  PortName=waves  Element=w_39
  waves_w_40 : Outport  Port=3  PortName=waves  Element=w_40
  waves_w_41 : Outport  Port=3  PortName=waves  Element=w_41
  waves_w_42 : Outport  Port=3  PortName=waves  Element=w_42
  waves_w_43 : Outport  Port=3  PortName=waves  Element=w_43
  waves_w_44 : Outport  Port=3  PortName=waves  Element=w_44
  waves_w_45 : Outport  Port=3  PortName=waves  Element=w_45
  waves_w_46 : Outport  Port=3  PortName=waves  Element=w_46
  waves_w_47 : Outport  Port=3  PortName=waves  Element=w_47
  waves_w_48 : Outport  Port=3  PortName=waves  Element=w_48
  waves_w_49 : Outport  Port=3  PortName=waves  Element=w_49
  waves_w_50 : Outport  Port=3  PortName=waves  Element=w_50
  waves_w_51 : Outport  Port=3  PortName=waves  Element=w_51
  waves_w_52 : Outport  Port=3  PortName=waves  Element=w_52
  waves_w_53 : Outport  Port=3  PortName=waves  Element=w_53
  waves_w_54 : Outport  Port=3  PortName=waves  Element=w_54
  wires:
  cfg_SA/1 -> SA/1
  SA/1 -> CellDelay_SA/1, Cells_c_SA/1
  CellDelay_SA/1 -> [c_SA]
  [gv_SA] -> SA/2
  cfg_SA_a/1 -> SA_a/1
  SA_a/1 -> CellDelay_SA_a/1, Cells_c_SA_a/1
  CellDelay_SA_a/1 -> [c_SA_a]
  [gv_SA_a] -> SA_a/2
  cfg_SA_b/1 -> SA_b/1
  SA_b/1 -> CellDelay_SA_b/1, Cells_c_SA_b/1
  CellDelay_SA_b/1 -> [c_SA_b]
  [gv_SA_b] -> SA_b/2
  cfg_SA_c/1 -> SA_c/1
  SA_c/1 -> CellDelay_SA_c/1, Cells_c_SA_c/1
  CellDelay_SA_c/1 -> [c_SA_c]
  [gv_SA_c] -> SA_c/2
  cfg_SA_d/1 -> SA_d/1
  SA_d/1 -> CellDelay_SA_d/1, Cells_c_SA_d/1
  CellDelay_SA_d/1 -> [c_SA_d]
  [gv_SA_d] -> SA_d/2
  cfg_CT/1 -> CT/1
  CT/1 -> CellDelay_CT/1, Cells_c_CT/1
  CellDelay_CT/1 -> [c_CT]
  [gv_CT] -> CT/2
  cfg_CT_a/1 -> CT_a/1
  CT_a/1 -> CellDelay_CT_a/1, Cells_c_CT_a/1
  CellDelay_CT_a/1 -> [c_CT_a]
  [gv_CT_a] -> CT_a/2
  cfg_OS/1 -> OS/1
  OS/1 -> CellDelay_OS/1, Cells_c_OS/1
  CellDelay_OS/1 -> [c_OS]
  [gv_OS] -> OS/2
  cfg_RE/1 -> RE/1
  RE/1 -> CellDelay_RE/1, Cells_c_RE/1
  CellDelay_RE/1 -> [c_RE]
  [gv_RE] -> RE/2
  cfg_LNB/1 -> LNB/1
  LNB/1 -> CellDelay_LNB/1, Cells_c_LNB/1
  CellDelay_LNB/1 -> [c_LNB]
  [gv_LNB] -> LNB/2
  cfg_TC_f/1 -> TC_f/1
  TC_f/1 -> CellDelay_TC_f/1, Cells_c_TC_f/1
  CellDelay_TC_f/1 -> [c_TC_f]
  [gv_TC_f] -> TC_f/2
  cfg_CN/1 -> CN/1
  CN/1 -> CellDelay_CN/1, Cells_c_CN/1
  CellDelay_CN/1 -> [c_CN]
  [gv_CN] -> CN/2
  cfg_RA_a/1 -> RA_a/1
  RA_a/1 -> CellDelay_RA_a/1, Cells_c_RA_a/1
  CellDelay_RA_a/1 -> [c_RA_a]
  [gv_RA_a] -> RA_a/2
  cfg_RA/1 -> RA/1
  RA/1 -> CellDelay_RA/1, Cells_c_RA/1
  CellDelay_RA/1 -> [c_RA]
  [gv_RA] -> RA/2
  cfg_CS_LA/1 -> CS_LA/1
  CS_LA/1 -> CellDelay_CS_LA/1, Cells_c_CS_LA/1
  CellDelay_CS_LA/1 -> [c_CS_LA]
  [gv_CS_LA] -> CS_LA/2
  cfg_Bach/1 -> Bach/1
  Bach/1 -> CellDelay_Bach/1, Cells_c_Bach/1
  CellDelay_Bach/1 -> [c_Bach]
  [gv_Bach] -> Bach/2
  cfg_LA_a/1 -> LA_a/1
  LA_a/1 -> CellDelay_LA_a/1, Cells_c_LA_a/1
  CellDelay_LA_a/1 -> [c_LA_a]
  [gv_LA_a] -> LA_a/2
  cfg_LA/1 -> LA/1
  LA/1 -> CellDelay_LA/1, Cells_c_LA/1
  CellDelay_LA/1 -> [c_LA]
  [gv_LA] -> LA/2
  cfg_BH/1 -> BH/1
  BH/1 -> CellDelay_BH/1, Cells_c_BH/1
  CellDelay_BH/1 -> [c_BH]
  [gv_BH] -> BH/2
  cfg_His_p/1 -> His_p/1
  His_p/1 -> CellDelay_His_p/1, Cells_c_His_p/1
  CellDelay_His_p/1 -> [c_His_p]
  [gv_His_p] -> His_p/2
  cfg_His_m/1 -> His_m/1
  His_m/1 -> CellDelay_His_m/1, Cells_c_His_m/1
  CellDelay_His_m/1 -> [c_His_m]
  [gv_His_m] -> His_m/2
  cfg_His_d/1 -> His_d/1
  His_d/1 -> CellDelay_His_d/1, Cells_c_His_d/1
  CellDelay_His_d/1 -> [c_His_d]
  [gv_His_d] -> His_d/2
  cfg_RBB_m/1 -> RBB_m/1
  RBB_m/1 -> CellDelay_RBB_m/1, Cells_c_RBB_m/1
  CellDelay_RBB_m/1 -> [c_RBB_m]
  [gv_RBB_m] -> RBB_m/2
  cfg_RBB/1 -> RBB/1
  RBB/1 -> CellDelay_RBB/1, Cells_c_RBB/1
  CellDelay_RBB/1 -> [c_RBB]
  [gv_RBB] -> RBB/2
  cfg_RBB_a/1 -> RBB_a/1
  RBB_a/1 -> CellDelay_RBB_a/1, Cells_c_RBB_a/1
  CellDelay_RBB_a/1 -> [c_RBB_a]
  [gv_RBB_a] -> RBB_a/2
  cfg_LBB_m/1 -> LBB_m/1
  LBB_m/1 -> CellDelay_LBB_m/1, Cells_c_LBB_m/1
  CellDelay_LBB_m/1 -> [c_LBB_m]
  [gv_LBB_m] -> LBB_m/2
  cfg_LBB/1 -> LBB/1
  LBB/1 -> CellDelay_LBB/1, Cells_c_LBB/1
  CellDelay_LBB/1 -> [c_LBB]
  [gv_LBB] -> LBB/2
  cfg_LBB_a/1 -> LBB_a/1
  LBB_a/1 -> CellDelay_LBB_a/1, Cells_c_LBB_a/1
  CellDelay_LBB_a/1 -> [c_LBB_a]
  [gv_LBB_a] -> LBB_a/2
  cfg_RVA/1 -> RVA/1
  RVA/1 -> CellDelay_RVA/1, Cells_c_RVA/1
  CellDelay_RVA/1 -> [c_RVA]
  [gv_RVA] -> RVA/2
  cfg_LVA/1 -> LVA/1
  LVA/1 -> CellDelay_LVA/1, Cells_c_LVA/1
  CellDelay_LVA/1 -> [c_LVA]
  [gv_LVA] -> LVA/2
  cfg_SEP_RV_m/1 -> SEP_RV_m/1
  SEP_RV_m/1 -> CellDelay_SEP_RV_m/1, Cells_c_SEP_RV_m/1
  CellDelay_SEP_RV_m/1 -> [c_SEP_RV_m]
  [gv_SEP_RV_m] -> SEP_RV_m/2
  cfg_SEP_RV/1 -> SEP_RV/1
  SEP_RV/1 -> CellDelay_SEP_RV/1, Cells_c_SEP_RV/1
  CellDelay_SEP_RV/1 -> [c_SEP_RV]
  [gv_SEP_RV] -> SEP_RV/2
  cfg_RV_m/1 -> RV_m/1
  RV_m/1 -> CellDelay_RV_m/1, Cells_c_RV_m/1
  CellDelay_RV_m/1 -> [c_RV_m]
  [gv_RV_m] -> RV_m/2
  cfg_RV/1 -> RV/1
  RV/1 -> CellDelay_RV/1, Cells_c_RV/1
  CellDelay_RV/1 -> [c_RV]
  [gv_RV] -> RV/2
  cfg_SEP_LV/1 -> SEP_LV/1
  SEP_LV/1 -> CellDelay_SEP_LV/1, Cells_c_SEP_LV/1
  CellDelay_SEP_LV/1 -> [c_SEP_LV]
  [gv_SEP_LV] -> SEP_LV/2
  cfg_CS_LV/1 -> CS_LV/1
  CS_LV/1 -> CellDelay_CS_LV/1, Cells_c_CS_LV/1
  CellDelay_CS_LV/1 -> [c_CS_LV]
  [gv_CS_LV] -> CS_LV/2
  cfg_SEP_LV_m/1 -> SEP_LV_m/1
  SEP_LV_m/1 -> CellDelay_SEP_LV_m/1, Cells_c_SEP_LV_m/1
  CellDelay_SEP_LV_m/1 -> [c_SEP_LV_m]
  [gv_SEP_LV_m] -> SEP_LV_m/2
  cfg_LV_m/1 -> LV_m/1
  LV_m/1 -> CellDelay_LV_m/1, Cells_c_LV_m/1
  CellDelay_LV_m/1 -> [c_LV_m]
  [gv_LV_m] -> LV_m/2
  cfg_LV/1 -> LV/1
  LV/1 -> CellDelay_LV/1, Cells_c_LV/1
  CellDelay_LV/1 -> [c_LV]
  [gv_LV] -> LV/2
  cfg_RV_mm/1 -> RV_mm/1
  RV_mm/1 -> CellDelay_RV_mm/1, Cells_c_RV_mm/1
  CellDelay_RV_mm/1 -> [c_RV_mm]
  [gv_RV_mm] -> RV_mm/2
  cfg_RVm/1 -> RVm/1
  RVm/1 -> CellDelay_RVm/1, Cells_c_RVm/1
  CellDelay_RVm/1 -> [c_RVm]
  [gv_RVm] -> RVm/2
  cfg_LV_mm/1 -> LV_mm/1
  LV_mm/1 -> CellDelay_LV_mm/1, Cells_c_LV_mm/1
  CellDelay_LV_mm/1 -> [c_LV_mm]
  [gv_LV_mm] -> LV_mm/2
  cfg_LVm/1 -> LVm/1
  LVm/1 -> CellDelay_LVm/1, Cells_c_LVm/1
  CellDelay_LVm/1 -> [c_LVm]
  [gv_LVm] -> LVm/2
  cfgPath_1_2/1 -> SA_SA_a/1
  SA_SA_a/1 -> [SA_a_J_SA_1]
  SA_SA_a/2 -> [SA_J_SA_a_1]
  SA_SA_a/3 -> [P_1]
  [c_SA] -> SA_SA_a/2
  [c_SA_a] -> SA_SA_a/3
  cfgPath_1_3/1 -> SA_SA_b/1
  SA_SA_b/1 -> [SA_b_J_SA_2]
  SA_SA_b/2 -> [SA_J_SA_b_2]
  SA_SA_b/3 -> [P_2]
  [c_SA] -> SA_SA_b/2
  [c_SA_b] -> SA_SA_b/3
  cfgPath_1_4/1 -> SA_SA_c/1
  SA_SA_c/1 -> [SA_c_J_SA_3]
  SA_SA_c/2 -> [SA_J_SA_c_3]
  SA_SA_c/3 -> [P_3]
  [c_SA] -> SA_SA_c/2
  [c_SA_c] -> SA_SA_c/3
  cfgPath_1_5/1 -> SA_SA_d/1
  SA_SA_d/1 -> [SA_d_J_SA_4]
  SA_SA_d/2 -> [SA_J_SA_d_4]
  SA_SA_d/3 -> [P_4]
  [c_SA] -> SA_SA_d/2
  [c_SA_d] -> SA_SA_d/3
  cfgPath_2_3/1 -> SA_a_SA_b/1
  SA_a_SA_b/1 -> [SA_b_J_SA_a_5]
  SA_a_SA_b/2 -> [SA_a_J_SA_b_5]
  SA_a_SA_b/3 -> [P_5]
  [c_SA_a] -> SA_a_SA_b/2
  [c_SA_b] -> SA_a_SA_b/3
  cfgPath_2_16/1 -> SA_a_Bach/1
  SA_a_Bach/1 -> [Bach_J_SA_a_6]
  SA_a_Bach/2 -> [SA_a_J_Bach_6]
  SA_a_Bach/3 -> [P_6]
  [c_SA_a] -> SA_a_Bach/2
  [c_Bach] -> SA_a_Bach/3
  cfgPath_3_4/1 -> SA_b_SA_c/1
  SA_b_SA_c/1 -> [SA_c_J_SA_b_7]
  SA_b_SA_c/2 -> [SA_b_J_SA_c_7]
  SA_b_SA_c/3 -> [P_7]
  [c_SA_b] -> SA_b_SA_c/2
  [c_SA_c] -> SA_b_SA_c/3
  cfgPath_3_13/1 -> SA_b_RA_a/1
  SA_b_RA_a/1 -> [RA_a_J_SA_b_8]
  SA_b_RA_a/2 -> [SA_b_J_RA_a_8]
  SA_b_RA_a/3 -> [P_8]
  [c_SA_b] -> SA_b_RA_a/2
  [c_RA_a] -> SA_b_RA_a/3
  cfgPath_4_5/1 -> SA_c_SA_d/1
  SA_c_SA_d/1 -> [SA_d_J_SA_c_9]
  SA_c_SA_d/2 -> [SA_c_J_SA_d_9]
  SA_c_SA_d/3 -> [P_9]
  [c_SA_c] -> SA_c_SA_d/2
  [c_SA_d] -> SA_c_SA_d/3
  cfgPath_4_8/1 -> SA_c_OS/1
  SA_c_OS/1 -> [OS_J_SA_c_10]
  SA_c_OS/2 -> [SA_c_J_OS_10]
  SA_c_OS/3 -> [P_10]
  [c_SA_c] -> SA_c_OS/2
  [c_OS] -> SA_c_OS/3
  cfgPath_5_7/1 -> SA_d_CT_a/1
  SA_d_CT_a/1 -> [CT_a_J_SA_d_11]
  SA_d_CT_a/2 -> [SA_d_J_CT_a_11]
  SA_d_CT_a/3 -> [P_11]
  [c_SA_d] -> SA_d_CT_a/2
  [c_CT_a] -> SA_d_CT_a/3
  cfgPath_6_7/1 -> CT_CT_a/1
  CT_CT_a/1 -> [CT_a_J_CT_12]
  CT_CT_a/2 -> [CT_J_CT_a_12]
  CT_CT_a/3 -> [P_12]
  [c_CT] -> CT_CT_a/2
  [c_CT_a] -> CT_CT_a/3
  cfgPath_8_9/1 -> OS_RE/1
  OS_RE/1 -> [RE_J_OS_13]
  OS_RE/2 -> [OS_J_RE_13]
  OS_RE/3 -> [P_13]
  [c_OS] -> OS_RE/2
  [c_RE] -> OS_RE/3
  cfgPath_8_11/1 -> OS_TC_f/1
  OS_TC_f/1 -> [TC_f_J_OS_14]
  OS_TC_f/2 -> [OS_J_TC_f_14]
  OS_TC_f/3 -> [P_14]
  [c_OS] -> OS_TC_f/2
  [c_TC_f] -> OS_TC_f/3
  cfgPath_9_10/1 -> RE_LNB/1
  RE_LNB/1 -> [LNB_J_RE_15]
  RE_LNB/2 -> [RE_J_LNB_15]
  RE_LNB/3 -> [P_15]
  [c_RE] -> RE_LNB/2
  [c_LNB] -> RE_LNB/3
  cfgPath_10_19/1 -> LNB_BH/1
  LNB_BH/1 -> [BH_J_LNB_16]
  LNB_BH/2 -> [LNB_J_BH_16]
  LNB_BH/3 -> [P_16]
  [c_LNB] -> LNB_BH/2
  [c_BH] -> LNB_BH/3
  cfgPath_11_12/1 -> TC_f_CN/1
  TC_f_CN/1 -> [CN_J_TC_f_17]
  TC_f_CN/2 -> [TC_f_J_CN_17]
  TC_f_CN/3 -> [P_17]
  [c_TC_f] -> TC_f_CN/2
  [c_CN] -> TC_f_CN/3
  cfgPath_12_19/1 -> CN_BH/1
  CN_BH/1 -> [BH_J_CN_18]
  CN_BH/2 -> [CN_J_BH_18]
  CN_BH/3 -> [P_18]
  [c_CN] -> CN_BH/2
  [c_BH] -> CN_BH/3
  cfgPath_13_14/1 -> RA_a_RA/1
  RA_a_RA/1 -> [RA_J_RA_a_19]
  RA_a_RA/2 -> [RA_a_J_RA_19]
  RA_a_RA/3 -> [P_19]
  [c_RA_a] -> RA_a_RA/2
  [c_RA] -> RA_a_RA/3
  cfgPath_14_15/1 -> RA_CS_LA/1
  RA_CS_LA/1 -> [CS_LA_J_RA_20]
  RA_CS_LA/2 -> [RA_J_CS_LA_20]
  RA_CS_LA/3 -> [P_20]
  [c_RA] -> RA_CS_LA/2
  [c_CS_LA] -> RA_CS_LA/3
  cfgPath_16_17/1 -> Bach_LA_a/1
  Bach_LA_a/1 -> [LA_a_J_Bach_21]
  Bach_LA_a/2 -> [Bach_J_LA_a_21]
  Bach_LA_a/3 -> [P_21]
  [c_Bach] -> Bach_LA_a/2
  [c_LA_a] -> Bach_LA_a/3
  cfgPath_17_18/1 -> LA_a_LA/1
  LA_a_LA/1 -> [LA_J_LA_a_22]
  LA_a_LA/2 -> [LA_a_J_LA_22]
  LA_a_LA/3 -> [P_22]
  [c_LA_a] -> LA_a_LA/2
  [c_LA] -> LA_a_LA/3
  cfgPath_19_20/1 -> BH_His_p/1
  BH_His_p/1 -> [His_p_J_BH_23]
  BH_His_p/2 -> [BH_J_His_p_23]
  BH_His_p/3 -> [P_23]
  [c_BH] -> BH_His_p/2
  [c_His_p] -> BH_His_p/3
  cfgPath_20_21/1 -> His_p_His_m/1
  His_p_His_m/1 -> [His_m_J_His_p_24]
  His_p_His_m/2 -> [His_p_J_His_m_24]
  His_p_His_m/3 -> [P_24]
  [c_His_p] -> His_p_His_m/2
  [c_His_m] -> His_p_His_m/3
  cfgPath_21_22/1 -> His_m_His_d/1
  His_m_His_d/1 -> [His_d_J_His_m_25]
  His_m_His_d/2 -> [His_m_J_His_d_25]
  His_m_His_d/3 -> [P_25]
  [c_His_m] -> His_m_His_d/2
  [c_His_d] -> His_m_His_d/3
  cfgPath_22_23/1 -> His_d_RBB_m/1
  His_d_RBB_m/1 -> [RBB_m_J_His_d_26]
  His_d_RBB_m/2 -> [His_d_J_RBB_m_26]
  His_d_RBB_m/3 -> [P_26]
  [c_His_d] -> His_d_RBB_m/2
  [c_RBB_m] -> His_d_RBB_m/3
  cfgPath_22_26/1 -> His_d_LBB_m/1
  His_d_LBB_m/1 -> [LBB_m_J_His_d_27]
  His_d_LBB_m/2 -> [His_d_J_LBB_m_27]
  His_d_LBB_m/3 -> [P_27]
  [c_His_d] -> His_d_LBB_m/2
  [c_LBB_m] -> His_d_LBB_m/3
  cfgPath_23_24/1 -> RBB_m_RBB/1
  RBB_m_RBB/1 -> [RBB_J_RBB_m_28]
  RBB_m_RBB/2 -> [RBB_m_J_RBB_28]
  RBB_m_RBB/3 -> [P_28]
  [c_RBB_m] -> RBB_m_RBB/2
  [c_RBB] -> RBB_m_RBB/3
  cfgPath_24_25/1 -> RBB_RBB_a/1
  RBB_RBB_a/1 -> [RBB_a_J_RBB_29]
  RBB_RBB_a/2 -> [RBB_J_RBB_a_29]
  RBB_RBB_a/3 -> [P_29]
  [c_RBB] -> RBB_RBB_a/2
  [c_RBB_a] -> RBB_RBB_a/3
  cfgPath_25_29/1 -> RBB_a_RVA/1
  RBB_a_RVA/1 -> [RVA_J_RBB_a_30]
  RBB_a_RVA/2 -> [RBB_a_J_RVA_30]
  RBB_a_RVA/3 -> [P_30]
  [c_RBB_a] -> RBB_a_RVA/2
  [c_RVA] -> RBB_a_RVA/3
  cfgPath_25_33/1 -> RBB_a_RV_m/1
  RBB_a_RV_m/1 -> [RV_m_J_RBB_a_31]
  RBB_a_RV_m/2 -> [RBB_a_J_RV_m_31]
  RBB_a_RV_m/3 -> [P_31]
  [c_RBB_a] -> RBB_a_RV_m/2
  [c_RV_m] -> RBB_a_RV_m/3
  cfgPath_26_27/1 -> LBB_m_LBB/1
  LBB_m_LBB/1 -> [LBB_J_LBB_m_32]
  LBB_m_LBB/2 -> [LBB_m_J_LBB_32]
  LBB_m_LBB/3 -> [P_32]
  [c_LBB_m] -> LBB_m_LBB/2
  [c_LBB] -> LBB_m_LBB/3
  cfgPath_26_37/1 -> LBB_m_SEP_LV_m/1
  LBB_m_SEP_LV_m/1 -> [SEP_LV_m_J_LBB_m_33]
  LBB_m_SEP_LV_m/2 -> [LBB_m_J_SEP_LV_m_33]
  LBB_m_SEP_LV_m/3 -> [P_33]
  [c_LBB_m] -> LBB_m_SEP_LV_m/2
  [c_SEP_LV_m] -> LBB_m_SEP_LV_m/3
  cfgPath_27_28/1 -> LBB_LBB_a/1
  LBB_LBB_a/1 -> [LBB_a_J_LBB_34]
  LBB_LBB_a/2 -> [LBB_J_LBB_a_34]
  LBB_LBB_a/3 -> [P_34]
  [c_LBB] -> LBB_LBB_a/2
  [c_LBB_a] -> LBB_LBB_a/3
  cfgPath_28_30/1 -> LBB_a_LVA/1
  LBB_a_LVA/1 -> [LVA_J_LBB_a_35]
  LBB_a_LVA/2 -> [LBB_a_J_LVA_35]
  LBB_a_LVA/3 -> [P_35]
  [c_LBB_a] -> LBB_a_LVA/2
  [c_LVA] -> LBB_a_LVA/3
  cfgPath_28_38/1 -> LBB_a_LV_m/1
  LBB_a_LV_m/1 -> [LV_m_J_LBB_a_36]
  LBB_a_LV_m/2 -> [LBB_a_J_LV_m_36]
  LBB_a_LV_m/3 -> [P_36]
  [c_LBB_a] -> LBB_a_LV_m/2
  [c_LV_m] -> LBB_a_LV_m/3
  cfgPath_29_30/1 -> RVA_LVA/1
  RVA_LVA/1 -> [LVA_J_RVA_37]
  RVA_LVA/2 -> [RVA_J_LVA_37]
  RVA_LVA/3 -> [P_37]
  [c_RVA] -> RVA_LVA/2
  [c_LVA] -> RVA_LVA/3
  cfgPath_29_31/1 -> RVA_SEP_RV_m/1
  RVA_SEP_RV_m/1 -> [SEP_RV_m_J_RVA_38]
  RVA_SEP_RV_m/2 -> [RVA_J_SEP_RV_m_38]
  RVA_SEP_RV_m/3 -> [P_38]
  [c_RVA] -> RVA_SEP_RV_m/2
  [c_SEP_RV_m] -> RVA_SEP_RV_m/3
  cfgPath_29_40/1 -> RVA_RV_mm/1
  RVA_RV_mm/1 -> [RV_mm_J_RVA_39]
  RVA_RV_mm/2 -> [RVA_J_RV_mm_39]
  RVA_RV_mm/3 -> [P_39]
  [c_RVA] -> RVA_RV_mm/2
  [c_RV_mm] -> RVA_RV_mm/3
  cfgPath_30_37/1 -> LVA_SEP_LV_m/1
  LVA_SEP_LV_m/1 -> [SEP_LV_m_J_LVA_40]
  LVA_SEP_LV_m/2 -> [LVA_J_SEP_LV_m_40]
  LVA_SEP_LV_m/3 -> [P_40]
  [c_LVA] -> LVA_SEP_LV_m/2
  [c_SEP_LV_m] -> LVA_SEP_LV_m/3
  cfgPath_30_42/1 -> LVA_LV_mm/1
  LVA_LV_mm/1 -> [LV_mm_J_LVA_41]
  LVA_LV_mm/2 -> [LVA_J_LV_mm_41]
  LVA_LV_mm/3 -> [P_41]
  [c_LVA] -> LVA_LV_mm/2
  [c_LV_mm] -> LVA_LV_mm/3
  cfgPath_31_32/1 -> SEP_RV_m_SEP_RV/1
  SEP_RV_m_SEP_RV/1 -> [SEP_RV_J_SEP_RV_m_42]
  SEP_RV_m_SEP_RV/2 -> [SEP_RV_m_J_SEP_RV_42]
  SEP_RV_m_SEP_RV/3 -> [P_42]
  [c_SEP_RV_m] -> SEP_RV_m_SEP_RV/2
  [c_SEP_RV] -> SEP_RV_m_SEP_RV/3
  cfgPath_31_37/1 -> SEP_RV_m_SEP_LV_m/1
  SEP_RV_m_SEP_LV_m/1 -> [SEP_LV_m_J_SEP_RV_m_43]
  SEP_RV_m_SEP_LV_m/2 -> [SEP_RV_m_J_SEP_LV_m_43]
  SEP_RV_m_SEP_LV_m/3 -> [P_43]
  [c_SEP_RV_m] -> SEP_RV_m_SEP_LV_m/2
  [c_SEP_LV_m] -> SEP_RV_m_SEP_LV_m/3
  cfgPath_32_35/1 -> SEP_RV_SEP_LV/1
  SEP_RV_SEP_LV/1 -> [SEP_LV_J_SEP_RV_44]
  SEP_RV_SEP_LV/2 -> [SEP_RV_J_SEP_LV_44]
  SEP_RV_SEP_LV/3 -> [P_44]
  [c_SEP_RV] -> SEP_RV_SEP_LV/2
  [c_SEP_LV] -> SEP_RV_SEP_LV/3
  cfgPath_33_34/1 -> RV_m_RV/1
  RV_m_RV/1 -> [RV_J_RV_m_45]
  RV_m_RV/2 -> [RV_m_J_RV_45]
  RV_m_RV/3 -> [P_45]
  [c_RV_m] -> RV_m_RV/2
  [c_RV] -> RV_m_RV/3
  cfgPath_33_40/1 -> RV_m_RV_mm/1
  RV_m_RV_mm/1 -> [RV_mm_J_RV_m_46]
  RV_m_RV_mm/2 -> [RV_m_J_RV_mm_46]
  RV_m_RV_mm/3 -> [P_46]
  [c_RV_m] -> RV_m_RV_mm/2
  [c_RV_mm] -> RV_m_RV_mm/3
  cfgPath_34_41/1 -> RV_RVm/1
  RV_RVm/1 -> [RVm_J_RV_47]
  RV_RVm/2 -> [RV_J_RVm_47]
  RV_RVm/3 -> [P_47]
  [c_RV] -> RV_RVm/2
  [c_RVm] -> RV_RVm/3
  cfgPath_35_36/1 -> SEP_LV_CS_LV/1
  SEP_LV_CS_LV/1 -> [CS_LV_J_SEP_LV_48]
  SEP_LV_CS_LV/2 -> [SEP_LV_J_CS_LV_48]
  SEP_LV_CS_LV/3 -> [P_48]
  [c_SEP_LV] -> SEP_LV_CS_LV/2
  [c_CS_LV] -> SEP_LV_CS_LV/3
  cfgPath_35_37/1 -> SEP_LV_SEP_LV_m/1
  SEP_LV_SEP_LV_m/1 -> [SEP_LV_m_J_SEP_LV_49]
  SEP_LV_SEP_LV_m/2 -> [SEP_LV_J_SEP_LV_m_49]
  SEP_LV_SEP_LV_m/3 -> [P_49]
  [c_SEP_LV] -> SEP_LV_SEP_LV_m/2
  [c_SEP_LV_m] -> SEP_LV_SEP_LV_m/3
  cfgPath_38_39/1 -> LV_m_LV/1
  LV_m_LV/1 -> [LV_J_LV_m_50]
  LV_m_LV/2 -> [LV_m_J_LV_50]
  LV_m_LV/3 -> [P_50]
  [c_LV_m] -> LV_m_LV/2
  [c_LV] -> LV_m_LV/3
  cfgPath_38_42/1 -> LV_m_LV_mm/1
  LV_m_LV_mm/1 -> [LV_mm_J_LV_m_51]
  LV_m_LV_mm/2 -> [LV_m_J_LV_mm_51]
  LV_m_LV_mm/3 -> [P_51]
  [c_LV_m] -> LV_m_LV_mm/2
  [c_LV_mm] -> LV_m_LV_mm/3
  cfgPath_39_43/1 -> LV_LVm/1
  LV_LVm/1 -> [LVm_J_LV_52]
  LV_LVm/2 -> [LV_J_LVm_52]
  LV_LVm/3 -> [P_52]
  [c_LV] -> LV_LVm/2
  [c_LVm] -> LV_LVm/3
  cfgPath_40_41/1 -> RV_mm_RVm/1
  RV_mm_RVm/1 -> [RVm_J_RV_mm_53]
  RV_mm_RVm/2 -> [RV_mm_J_RVm_53]
  RV_mm_RVm/3 -> [P_53]
  [c_RV_mm] -> RV_mm_RVm/2
  [c_RVm] -> RV_mm_RVm/3
  cfgPath_42_43/1 -> LV_mm_LVm/1
  LV_mm_LVm/1 -> [LVm_J_LV_mm_54]
  LV_mm_LVm/2 -> [LV_mm_J_LVm_54]
  LV_mm_LVm/3 -> [P_54]
  [c_LV_mm] -> LV_mm_LVm/2
  [c_LVm] -> LV_mm_LVm/3
  [P_1] -> SA_SA_a_probe/1
  [Leads] -> SA_SA_a_probe/2
  [P_2] -> SA_SA_b_probe/1
  [Leads] -> SA_SA_b_probe/2
  [P_3] -> SA_SA_c_probe/1
  [Leads] -> SA_SA_c_probe/2
  [P_4] -> SA_SA_d_probe/1
  [Leads] -> SA_SA_d_probe/2
  [P_5] -> SA_a_SA_b_probe/1
  [Leads] -> SA_a_SA_b_probe/2
  [P_6] -> SA_a_Bach_probe/1
  [Leads] -> SA_a_Bach_probe/2
  [P_7] -> SA_b_SA_c_probe/1
  [Leads] -> SA_b_SA_c_probe/2
  [P_8] -> SA_b_RA_a_probe/1
  [Leads] -> SA_b_RA_a_probe/2
  [P_9] -> SA_c_SA_d_probe/1
  [Leads] -> SA_c_SA_d_probe/2
  [P_10] -> SA_c_OS_probe/1
  [Leads] -> SA_c_OS_probe/2
  [P_11] -> SA_d_CT_a_probe/1
  [Leads] -> SA_d_CT_a_probe/2
  [P_12] -> CT_CT_a_probe/1
  [Leads] -> CT_CT_a_probe/2
  [P_13] -> OS_RE_probe/1
  [Leads] -> OS_RE_probe/2
  [P_14] -> OS_TC_f_probe/1
  [Leads] -> OS_TC_f_probe/2
  [P_15] -> RE_LNB_probe/1
  [Leads] -> RE_LNB_probe/2
  [P_16] -> LNB_BH_probe/1
  [Leads] -> LNB_BH_probe/2
  [P_17] -> TC_f_CN_probe/1
  [Leads] -> TC_f_CN_probe/2
  [P_18] -> CN_BH_probe/1
  [Leads] -> CN_BH_probe/2
  [P_19] -> RA_a_RA_probe/1
  [Leads] -> RA_a_RA_probe/2
  [P_20] -> RA_CS_LA_probe/1
  [Leads] -> RA_CS_LA_probe/2
  [P_21] -> Bach_LA_a_probe/1
  [Leads] -> Bach_LA_a_probe/2
  [P_22] -> LA_a_LA_probe/1
  [Leads] -> LA_a_LA_probe/2
  [P_23] -> BH_His_p_probe/1
  [Leads] -> BH_His_p_probe/2
  [P_24] -> His_p_His_m_probe/1
  [Leads] -> His_p_His_m_probe/2
  [P_25] -> His_m_His_d_probe/1
  [Leads] -> His_m_His_d_probe/2
  [P_26] -> His_d_RBB_m_probe/1
  [Leads] -> His_d_RBB_m_probe/2
  [P_27] -> His_d_LBB_m_probe/1
  [Leads] -> His_d_LBB_m_probe/2
  [P_28] -> RBB_m_RBB_probe/1
  [Leads] -> RBB_m_RBB_probe/2
  [P_29] -> RBB_RBB_a_probe/1
  [Leads] -> RBB_RBB_a_probe/2
  [P_30] -> RBB_a_RVA_probe/1
  [Leads] -> RBB_a_RVA_probe/2
  [P_31] -> RBB_a_RV_m_probe/1
  [Leads] -> RBB_a_RV_m_probe/2
  [P_32] -> LBB_m_LBB_probe/1
  [Leads] -> LBB_m_LBB_probe/2
  [P_33] -> LBB_m_SEP_LV_m_probe/1
  [Leads] -> LBB_m_SEP_LV_m_probe/2
  [P_34] -> LBB_LBB_a_probe/1
  [Leads] -> LBB_LBB_a_probe/2
  [P_35] -> LBB_a_LVA_probe/1
  [Leads] -> LBB_a_LVA_probe/2
  [P_36] -> LBB_a_LV_m_probe/1
  [Leads] -> LBB_a_LV_m_probe/2
  [P_37] -> RVA_LVA_probe/1
  [Leads] -> RVA_LVA_probe/2
  [P_38] -> RVA_SEP_RV_m_probe/1
  [Leads] -> RVA_SEP_RV_m_probe/2
  [P_39] -> RVA_RV_mm_probe/1
  [Leads] -> RVA_RV_mm_probe/2
  [P_40] -> LVA_SEP_LV_m_probe/1
  [Leads] -> LVA_SEP_LV_m_probe/2
  [P_41] -> LVA_LV_mm_probe/1
  [Leads] -> LVA_LV_mm_probe/2
  [P_42] -> SEP_RV_m_SEP_RV_probe/1
  [Leads] -> SEP_RV_m_SEP_RV_probe/2
  [P_43] -> SEP_RV_m_SEP_LV_m_probe/1
  [Leads] -> SEP_RV_m_SEP_LV_m_probe/2
  [P_44] -> SEP_RV_SEP_LV_probe/1
  [Leads] -> SEP_RV_SEP_LV_probe/2
  [P_45] -> RV_m_RV_probe/1
  [Leads] -> RV_m_RV_probe/2
  [P_46] -> RV_m_RV_mm_probe/1
  [Leads] -> RV_m_RV_mm_probe/2
  [P_47] -> RV_RVm_probe/1
  [Leads] -> RV_RVm_probe/2
  [P_48] -> SEP_LV_CS_LV_probe/1
  [Leads] -> SEP_LV_CS_LV_probe/2
  [P_49] -> SEP_LV_SEP_LV_m_probe/1
  [Leads] -> SEP_LV_SEP_LV_m_probe/2
  [P_50] -> LV_m_LV_probe/1
  [Leads] -> LV_m_LV_probe/2
  [P_51] -> LV_m_LV_mm_probe/1
  [Leads] -> LV_m_LV_mm_probe/2
  [P_52] -> LV_LVm_probe/1
  [Leads] -> LV_LVm_probe/2
  [P_53] -> RV_mm_RVm_probe/1
  [Leads] -> RV_mm_RVm_probe/2
  [P_54] -> LV_mm_LVm_probe/1
  [Leads] -> LV_mm_LVm_probe/2
  [SA_a_J_SA_1] -> Node1_OR/1
  [SA_b_J_SA_2] -> Node1_OR/2
  [SA_c_J_SA_3] -> Node1_OR/3
  [SA_d_J_SA_4] -> Node1_OR/4
  Node1_OR/1 -> [gv_SA]
  [SA_J_SA_a_1] -> Node2_OR/1
  [SA_b_J_SA_a_5] -> Node2_OR/2
  [Bach_J_SA_a_6] -> Node2_OR/3
  Node2_OR/1 -> [gv_SA_a]
  [SA_J_SA_b_2] -> Node3_OR/1
  [SA_a_J_SA_b_5] -> Node3_OR/2
  [SA_c_J_SA_b_7] -> Node3_OR/3
  [RA_a_J_SA_b_8] -> Node3_OR/4
  Node3_OR/1 -> [gv_SA_b]
  [SA_J_SA_c_3] -> Node4_OR/1
  [SA_b_J_SA_c_7] -> Node4_OR/2
  [SA_d_J_SA_c_9] -> Node4_OR/3
  [OS_J_SA_c_10] -> Node4_OR/4
  Node4_OR/1 -> [gv_SA_c]
  [SA_J_SA_d_4] -> Node5_OR/1
  [SA_c_J_SA_d_9] -> Node5_OR/2
  [CT_a_J_SA_d_11] -> Node5_OR/3
  Node5_OR/1 -> [gv_SA_d]
  [CT_a_J_CT_12] -> [gv_CT]
  [SA_d_J_CT_a_11] -> Node7_OR/1
  [CT_J_CT_a_12] -> Node7_OR/2
  Node7_OR/1 -> [gv_CT_a]
  [SA_c_J_OS_10] -> Node8_OR/1
  [RE_J_OS_13] -> Node8_OR/2
  [TC_f_J_OS_14] -> Node8_OR/3
  Node8_OR/1 -> [gv_OS]
  [OS_J_RE_13] -> Node9_OR/1
  [LNB_J_RE_15] -> Node9_OR/2
  Node9_OR/1 -> [gv_RE]
  [RE_J_LNB_15] -> Node10_OR/1
  [BH_J_LNB_16] -> Node10_OR/2
  Node10_OR/1 -> [gv_LNB]
  [OS_J_TC_f_14] -> Node11_OR/1
  [CN_J_TC_f_17] -> Node11_OR/2
  Node11_OR/1 -> [gv_TC_f]
  [TC_f_J_CN_17] -> Node12_OR/1
  [BH_J_CN_18] -> Node12_OR/2
  Node12_OR/1 -> [gv_CN]
  [SA_b_J_RA_a_8] -> Node13_OR/1
  [RA_J_RA_a_19] -> Node13_OR/2
  Node13_OR/1 -> [gv_RA_a]
  [RA_a_J_RA_19] -> Node14_OR/1
  [CS_LA_J_RA_20] -> Node14_OR/2
  [AP] -> Node14_OR/3
  Node14_OR/1 -> [gv_RA]
  [RA_J_CS_LA_20] -> [gv_CS_LA]
  [SA_a_J_Bach_6] -> Node16_OR/1
  [LA_a_J_Bach_21] -> Node16_OR/2
  Node16_OR/1 -> [gv_Bach]
  [Bach_J_LA_a_21] -> Node17_OR/1
  [LA_J_LA_a_22] -> Node17_OR/2
  Node17_OR/1 -> [gv_LA_a]
  [LA_a_J_LA_22] -> [gv_LA]
  [LNB_J_BH_16] -> Node19_OR/1
  [CN_J_BH_18] -> Node19_OR/2
  [His_p_J_BH_23] -> Node19_OR/3
  Node19_OR/1 -> [gv_BH]
  [BH_J_His_p_23] -> Node20_OR/1
  [His_m_J_His_p_24] -> Node20_OR/2
  Node20_OR/1 -> [gv_His_p]
  [His_p_J_His_m_24] -> Node21_OR/1
  [His_d_J_His_m_25] -> Node21_OR/2
  Node21_OR/1 -> [gv_His_m]
  [His_m_J_His_d_25] -> Node22_OR/1
  [RBB_m_J_His_d_26] -> Node22_OR/2
  [LBB_m_J_His_d_27] -> Node22_OR/3
  Node22_OR/1 -> [gv_His_d]
  [His_d_J_RBB_m_26] -> Node23_OR/1
  [RBB_J_RBB_m_28] -> Node23_OR/2
  Node23_OR/1 -> [gv_RBB_m]
  [RBB_m_J_RBB_28] -> Node24_OR/1
  [RBB_a_J_RBB_29] -> Node24_OR/2
  Node24_OR/1 -> [gv_RBB]
  [RBB_J_RBB_a_29] -> Node25_OR/1
  [RVA_J_RBB_a_30] -> Node25_OR/2
  [RV_m_J_RBB_a_31] -> Node25_OR/3
  Node25_OR/1 -> [gv_RBB_a]
  [His_d_J_LBB_m_27] -> Node26_OR/1
  [LBB_J_LBB_m_32] -> Node26_OR/2
  [SEP_LV_m_J_LBB_m_33] -> Node26_OR/3
  Node26_OR/1 -> [gv_LBB_m]
  [LBB_m_J_LBB_32] -> Node27_OR/1
  [LBB_a_J_LBB_34] -> Node27_OR/2
  Node27_OR/1 -> [gv_LBB]
  [LBB_J_LBB_a_34] -> Node28_OR/1
  [LVA_J_LBB_a_35] -> Node28_OR/2
  [LV_m_J_LBB_a_36] -> Node28_OR/3
  Node28_OR/1 -> [gv_LBB_a]
  [RBB_a_J_RVA_30] -> Node29_OR/1
  [LVA_J_RVA_37] -> Node29_OR/2
  [SEP_RV_m_J_RVA_38] -> Node29_OR/3
  [RV_mm_J_RVA_39] -> Node29_OR/4
  [VP] -> Node29_OR/5
  Node29_OR/1 -> [gv_RVA]
  [LBB_a_J_LVA_35] -> Node30_OR/1
  [RVA_J_LVA_37] -> Node30_OR/2
  [SEP_LV_m_J_LVA_40] -> Node30_OR/3
  [LV_mm_J_LVA_41] -> Node30_OR/4
  Node30_OR/1 -> [gv_LVA]
  [RVA_J_SEP_RV_m_38] -> Node31_OR/1
  [SEP_RV_J_SEP_RV_m_42] -> Node31_OR/2
  [SEP_LV_m_J_SEP_RV_m_43] -> Node31_OR/3
  Node31_OR/1 -> [gv_SEP_RV_m]
  [SEP_RV_m_J_SEP_RV_42] -> Node32_OR/1
  [SEP_LV_J_SEP_RV_44] -> Node32_OR/2
  Node32_OR/1 -> [gv_SEP_RV]
  [RBB_a_J_RV_m_31] -> Node33_OR/1
  [RV_J_RV_m_45] -> Node33_OR/2
  [RV_mm_J_RV_m_46] -> Node33_OR/3
  Node33_OR/1 -> [gv_RV_m]
  [RV_m_J_RV_45] -> Node34_OR/1
  [RVm_J_RV_47] -> Node34_OR/2
  Node34_OR/1 -> [gv_RV]
  [SEP_RV_J_SEP_LV_44] -> Node35_OR/1
  [CS_LV_J_SEP_LV_48] -> Node35_OR/2
  [SEP_LV_m_J_SEP_LV_49] -> Node35_OR/3
  Node35_OR/1 -> [gv_SEP_LV]
  [SEP_LV_J_CS_LV_48] -> [gv_CS_LV]
  [LBB_m_J_SEP_LV_m_33] -> Node37_OR/1
  [LVA_J_SEP_LV_m_40] -> Node37_OR/2
  [SEP_RV_m_J_SEP_LV_m_43] -> Node37_OR/3
  [SEP_LV_J_SEP_LV_m_49] -> Node37_OR/4
  Node37_OR/1 -> [gv_SEP_LV_m]
  [LBB_a_J_LV_m_36] -> Node38_OR/1
  [LV_J_LV_m_50] -> Node38_OR/2
  [LV_mm_J_LV_m_51] -> Node38_OR/3
  Node38_OR/1 -> [gv_LV_m]
  [LV_m_J_LV_50] -> Node39_OR/1
  [LVm_J_LV_52] -> Node39_OR/2
  Node39_OR/1 -> [gv_LV]
  [RVA_J_RV_mm_39] -> Node40_OR/1
  [RV_m_J_RV_mm_46] -> Node40_OR/2
  [RVm_J_RV_mm_53] -> Node40_OR/3
  Node40_OR/1 -> [gv_RV_mm]
  [RV_J_RVm_47] -> Node41_OR/1
  [RV_mm_J_RVm_53] -> Node41_OR/2
  Node41_OR/1 -> [gv_RVm]
  [LVA_J_LV_mm_41] -> Node42_OR/1
  [LV_m_J_LV_mm_51] -> Node42_OR/2
  [LVm_J_LV_mm_54] -> Node42_OR/3
  Node42_OR/1 -> [gv_LV_mm]
  [LV_J_LVm_52] -> Node43_OR/1
  [LV_mm_J_LVm_54] -> Node43_OR/2
  Node43_OR/1 -> [gv_LVm]
  Leads/1 -> [Leads]
  Pace/1 -> Pacing/1
  Pacing/1 -> [AP]
  Pacing/2 -> [VP]
  SA_SA_a_probe/1 -> [EGM_1]
  SA_SA_a_probe/2 -> waves_w_1/1
  SA_SA_b_probe/1 -> [EGM_2]
  SA_SA_b_probe/2 -> waves_w_2/1
  SA_SA_c_probe/1 -> [EGM_3]
  SA_SA_c_probe/2 -> waves_w_3/1
  SA_SA_d_probe/1 -> [EGM_4]
  SA_SA_d_probe/2 -> waves_w_4/1
  SA_a_SA_b_probe/1 -> [EGM_5]
  SA_a_SA_b_probe/2 -> waves_w_5/1
  SA_a_Bach_probe/1 -> [EGM_6]
  SA_a_Bach_probe/2 -> waves_w_6/1
  SA_b_SA_c_probe/1 -> [EGM_7]
  SA_b_SA_c_probe/2 -> waves_w_7/1
  SA_b_RA_a_probe/1 -> [EGM_8]
  SA_b_RA_a_probe/2 -> waves_w_8/1
  SA_c_SA_d_probe/1 -> [EGM_9]
  SA_c_SA_d_probe/2 -> waves_w_9/1
  SA_c_OS_probe/1 -> [EGM_10]
  SA_c_OS_probe/2 -> waves_w_10/1
  SA_d_CT_a_probe/1 -> [EGM_11]
  SA_d_CT_a_probe/2 -> waves_w_11/1
  CT_CT_a_probe/1 -> [EGM_12]
  CT_CT_a_probe/2 -> waves_w_12/1
  OS_RE_probe/1 -> [EGM_13]
  OS_RE_probe/2 -> waves_w_13/1
  OS_TC_f_probe/1 -> [EGM_14]
  OS_TC_f_probe/2 -> waves_w_14/1
  RE_LNB_probe/1 -> [EGM_15]
  RE_LNB_probe/2 -> waves_w_15/1
  LNB_BH_probe/1 -> [EGM_16]
  LNB_BH_probe/2 -> waves_w_16/1
  TC_f_CN_probe/1 -> [EGM_17]
  TC_f_CN_probe/2 -> waves_w_17/1
  CN_BH_probe/1 -> [EGM_18]
  CN_BH_probe/2 -> waves_w_18/1
  RA_a_RA_probe/1 -> [EGM_19]
  RA_a_RA_probe/2 -> waves_w_19/1
  RA_CS_LA_probe/1 -> [EGM_20]
  RA_CS_LA_probe/2 -> waves_w_20/1
  Bach_LA_a_probe/1 -> [EGM_21]
  Bach_LA_a_probe/2 -> waves_w_21/1
  LA_a_LA_probe/1 -> [EGM_22]
  LA_a_LA_probe/2 -> waves_w_22/1
  BH_His_p_probe/1 -> [EGM_23]
  BH_His_p_probe/2 -> waves_w_23/1
  His_p_His_m_probe/1 -> [EGM_24]
  His_p_His_m_probe/2 -> waves_w_24/1
  His_m_His_d_probe/1 -> [EGM_25]
  His_m_His_d_probe/2 -> waves_w_25/1
  His_d_RBB_m_probe/1 -> [EGM_26]
  His_d_RBB_m_probe/2 -> waves_w_26/1
  His_d_LBB_m_probe/1 -> [EGM_27]
  His_d_LBB_m_probe/2 -> waves_w_27/1
  RBB_m_RBB_probe/1 -> [EGM_28]
  RBB_m_RBB_probe/2 -> waves_w_28/1
  RBB_RBB_a_probe/1 -> [EGM_29]
  RBB_RBB_a_probe/2 -> waves_w_29/1
  RBB_a_RVA_probe/1 -> [EGM_30]
  RBB_a_RVA_probe/2 -> waves_w_30/1
  RBB_a_RV_m_probe/1 -> [EGM_31]
  RBB_a_RV_m_probe/2 -> waves_w_31/1
  LBB_m_LBB_probe/1 -> [EGM_32]
  LBB_m_LBB_probe/2 -> waves_w_32/1
  LBB_m_SEP_LV_m_probe/1 -> [EGM_33]
  LBB_m_SEP_LV_m_probe/2 -> waves_w_33/1
  LBB_LBB_a_probe/1 -> [EGM_34]
  LBB_LBB_a_probe/2 -> waves_w_34/1
  LBB_a_LVA_probe/1 -> [EGM_35]
  LBB_a_LVA_probe/2 -> waves_w_35/1
  LBB_a_LV_m_probe/1 -> [EGM_36]
  LBB_a_LV_m_probe/2 -> waves_w_36/1
  RVA_LVA_probe/1 -> [EGM_37]
  RVA_LVA_probe/2 -> waves_w_37/1
  RVA_SEP_RV_m_probe/1 -> [EGM_38]
  RVA_SEP_RV_m_probe/2 -> waves_w_38/1
  RVA_RV_mm_probe/1 -> [EGM_39]
  RVA_RV_mm_probe/2 -> waves_w_39/1
  LVA_SEP_LV_m_probe/1 -> [EGM_40]
  LVA_SEP_LV_m_probe/2 -> waves_w_40/1
  LVA_LV_mm_probe/1 -> [EGM_41]
  LVA_LV_mm_probe/2 -> waves_w_41/1
  SEP_RV_m_SEP_RV_probe/1 -> [EGM_42]
  SEP_RV_m_SEP_RV_probe/2 -> waves_w_42/1
  SEP_RV_m_SEP_LV_m_probe/1 -> [EGM_43]
  SEP_RV_m_SEP_LV_m_probe/2 -> waves_w_43/1
  SEP_RV_SEP_LV_probe/1 -> [EGM_44]
  SEP_RV_SEP_LV_probe/2 -> waves_w_44/1
  RV_m_RV_probe/1 -> [EGM_45]
  RV_m_RV_probe/2 -> waves_w_45/1
  RV_m_RV_mm_probe/1 -> [EGM_46]
  RV_m_RV_mm_probe/2 -> waves_w_46/1
  RV_RVm_probe/1 -> [EGM_47]
  RV_RVm_probe/2 -> waves_w_47/1
  SEP_LV_CS_LV_probe/1 -> [EGM_48]
  SEP_LV_CS_LV_probe/2 -> waves_w_48/1
  SEP_LV_SEP_LV_m_probe/1 -> [EGM_49]
  SEP_LV_SEP_LV_m_probe/2 -> waves_w_49/1
  LV_m_LV_probe/1 -> [EGM_50]
  LV_m_LV_probe/2 -> waves_w_50/1
  LV_m_LV_mm_probe/1 -> [EGM_51]
  LV_m_LV_mm_probe/2 -> waves_w_51/1
  LV_LVm_probe/1 -> [EGM_52]
  LV_LVm_probe/2 -> waves_w_52/1
  RV_mm_RVm_probe/1 -> [EGM_53]
  RV_mm_RVm_probe/2 -> waves_w_53/1
  LV_mm_LVm_probe/1 -> [EGM_54]
  LV_mm_LVm_probe/2 -> waves_w_54/1
  [EGM_1] -> EGMs_Sum/1
  [EGM_2] -> EGMs_Sum/2
  [EGM_3] -> EGMs_Sum/3
  [EGM_4] -> EGMs_Sum/4
  [EGM_5] -> EGMs_Sum/5
  [EGM_6] -> EGMs_Sum/6
  [EGM_7] -> EGMs_Sum/7
  [EGM_8] -> EGMs_Sum/8
  [EGM_9] -> EGMs_Sum/9
  [EGM_10] -> EGMs_Sum/10
  [EGM_11] -> EGMs_Sum/11
  [EGM_12] -> EGMs_Sum/12
  [EGM_13] -> EGMs_Sum/13
  [EGM_14] -> EGMs_Sum/14
  [EGM_15] -> EGMs_Sum/15
  [EGM_16] -> EGMs_Sum/16
  [EGM_17] -> EGMs_Sum/17
  [EGM_18] -> EGMs_Sum/18
  [EGM_19] -> EGMs_Sum/19
  [EGM_20] -> EGMs_Sum/20
  [EGM_21] -> EGMs_Sum/21
  [EGM_22] -> EGMs_Sum/22
  [EGM_23] -> EGMs_Sum/23
  [EGM_24] -> EGMs_Sum/24
  [EGM_25] -> EGMs_Sum/25
  [EGM_26] -> EGMs_Sum/26
  [EGM_27] -> EGMs_Sum/27
  [EGM_28] -> EGMs_Sum/28
  [EGM_29] -> EGMs_Sum/29
  [EGM_30] -> EGMs_Sum/30
  [EGM_31] -> EGMs_Sum/31
  [EGM_32] -> EGMs_Sum/32
  [EGM_33] -> EGMs_Sum/33
  [EGM_34] -> EGMs_Sum/34
  [EGM_35] -> EGMs_Sum/35
  [EGM_36] -> EGMs_Sum/36
  [EGM_37] -> EGMs_Sum/37
  [EGM_38] -> EGMs_Sum/38
  [EGM_39] -> EGMs_Sum/39
  [EGM_40] -> EGMs_Sum/40
  [EGM_41] -> EGMs_Sum/41
  [EGM_42] -> EGMs_Sum/42
  [EGM_43] -> EGMs_Sum/43
  [EGM_44] -> EGMs_Sum/44
  [EGM_45] -> EGMs_Sum/45
  [EGM_46] -> EGMs_Sum/46
  [EGM_47] -> EGMs_Sum/47
  [EGM_48] -> EGMs_Sum/48
  [EGM_49] -> EGMs_Sum/49
  [EGM_50] -> EGMs_Sum/50
  [EGM_51] -> EGMs_Sum/51
  [EGM_52] -> EGMs_Sum/52
  [EGM_53] -> EGMs_Sum/53
  [EGM_54] -> EGMs_Sum/54
  EGMs_Sum/1 -> EGMs/1
